simulink library "bcm"  (R2021b)
settings: Solver=VariableStepAuto  StartTime=0.0  StopTime=10.0  RelTol=1e-3
undefined symbols (not defined in the file or in its folder): ENUM_ANTITHEFT_ALARM, ENUM_ANTITHEFT_ARM, ENUM_ANTITHEFT_DISARM, ENUM_ANTITHEFT_WAIT, ENUM_GEARPOSNTOCAN_P, ENUM_PDKEYRAWLULOCK_INUNLOCK, ENUM_PDKEYRAWPS_INPS, ENUM_POWERSTA_ON, ENUM_POWERSTA_READY, ENUM_POWERSTA_STANDBY, ENUM_PWRSTASW_ON, ENUM_PWRSTASW_READY, ENUM_VEHICLETYPE_D21, ENUM_VEHICLETYPE_D31F25, ENUM_VEHICLETYPE_D31HAWD, ENUM_VEHICLETYPE_D31HRWD, ENUM_VEHICLETYPE_D31L24, FALSE, KBCM_ACCSwcPrsTmr_s, KBCM_ALMBrightnessDark_enum, KBCM_AmbBlue_enum, KBCM_AmbBreathT_ms, KBCM_AmbGreen_enum, KBCM_AmbMidPple_enum, KBCM_AmbRed_enum, KBCM_AmbTempCtrlEN_flg, KBCM_AmbTempT_s, KBCM_AmbWelModeENWait_s, KBCM_Antitheft_enum_ovrdflg, KBCM_Antitheft_enum_ovrdval, KBCM_APMDoorCtrlSta_flg_ovrdflg, KBCM_APMDoorCtrlSta_flg_ovrdval, KBCM_CmdKeepT_s, KBCM_CSWLightRstDebT_s, KBCM_CSWTurnLPRstT_s, KBCM_DelayTSW_flg, KBCM_DiagDRLOFF_flg, KBCM_DiagFLTC_mA, KBCM_DiagFMHT_s, KBCM_DiagFRTC_mA, KBCM_DiagRLTC_mA, KBCM_DiagRRTC_mA, KBCM_DrAPMRetryTimes_cnt, KBCM_DrOpenWdwOT_s, KBCM_DrOpenWdwReady_s, KBCM_ESSOffT_ms, KBCM_ESSOnT_ms, KBCM_FDCDKCReDetectT_K, KBCM_FDCDKCUSSFilterT_K, KBCM_HandleLampKeepT_s, KBCM_IVIRstHoldT_ms, KBCM_IVIRstTriggerT_ms, KBCM_ONDelayT_ms, KBCM_RAPSAbnFlashOFFT_ms, KBCM_RAPSAbnFlashONT_ms, KBCM_ReDetectT_K, KBCM_RightHandDriveEN_flg, KBCM_RLSLowSpdFilterT_s, KBCM_RmLampKeep_min, KBCM_RmLpKeyInT_s ... (+37)
libraries: simulink x447, $bdroot x11, hcu_lib x2
(part 2 of 13)

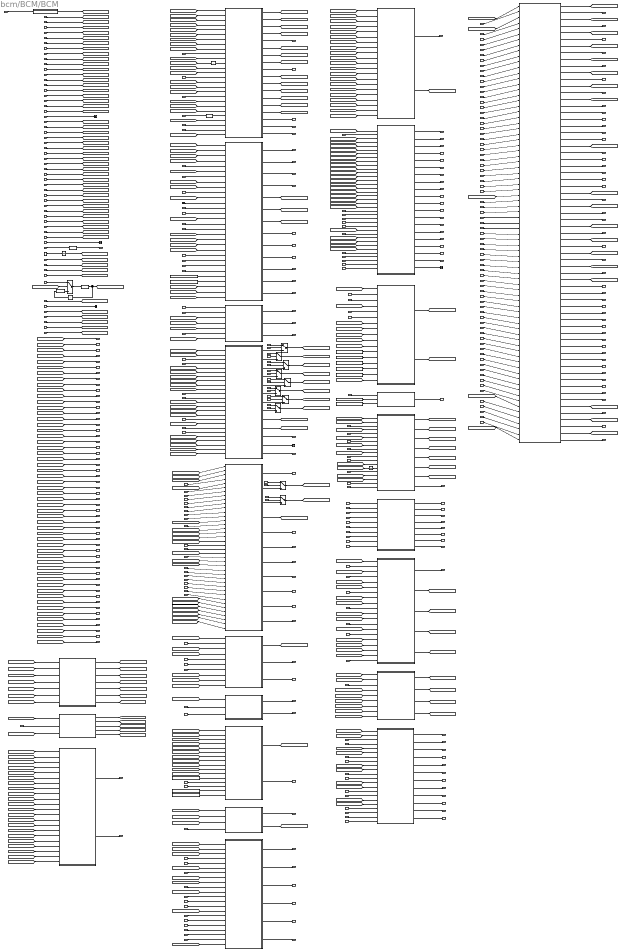
== system bcm/BCM/BCM ==
  task_time_s : Inport
  VINP_VehSpeed_kph : Inport  Port=2
  VINP_AirBagFailCmd_flg : Inport  Port=3
  VINP_ActBrkLampSta_flg : Inport  Port=4
  VINP_ESSActive_flg : Inport  Port=5
  VINP_SASAngle_Deg : Inport  Port=6
  VINP_SRRBSDWarnR_enum : Inport  Port=7
  VINP_SRRBSDWarnL_enum : Inport  Port=8
  VINP_LeftTurnReq_flg : Inport  Port=9
  VINP_RightTurnReq_flg : Inport  Port=10
  VINP_ForceLowBeam_enum : Inport  Port=11
  VINP_HazardWarningReq_flg : Inport  Port=12
  VINP_ADASACCSta_enum : Inport  Port=13
  VINP_TimeGapLevel_enum : Inport  Port=14
  VINP_SRRODASoundL_flg : Inport  Port=15
  VINP_SRRODASoundR_flg : Inport  Port=16
  VINP_SRRODAWarnL_enum : Inport  Port=17
  VINP_SRRODAWarnR_enum : Inport  Port=18
  VINP_SetUnlockSingle_flg : Inport  Port=19
  VINP_IVIStatus_flg : Inport  Port=20
  VINP_IVINightModeSta_flg : Inport  Port=21
  VINP_HeadLampSW_enum : Inport  Port=22
  VINP_RFogLampSW_flg : Inport  Port=23
  VINP_FollowMeSW_flg : Inport  Port=24
  VINP_IVIRRDefReq_flg : Inport  Port=25
  VINP_IVIWIMAINSW_flg : Inport  Port=26
  VINP_CANMsgValidIVI2_flg : Inport  Port=27
  VINP_CDLUnlockButt_flg : Inport  Port=28  OutDataTypeStr=boolean
  VINP_CDLLockButt_flg : Inport  Port=29  OutDataTypeStr=boolean
  VINP_RoomLampMode_flg : Inport  Port=30
  VINP_MFRDNBrightReq_pct : Inport  Port=31
  VINP_METERKPHCalcu_kph : Inport  Port=32
  VINP_IVIPWModeReq_enum : Inport  Port=33
  VINP_AmbLighLowBatAlertSW_flg : Inport  Port=34
  VINP_AmbLighSafetyAlertSW_flg : Inport  Port=35
  VINP_AmbLightBrightnessSet_enum : Inport  Port=36
  VINP_AmbLightDimInDarkSW_flg : Inport  Port=37
  VINP_AmbLightSW_flg : Inport  Port=38
  VINP_AmbLightWlcmLightSW_flg : Inport  Port=39
  VINP_LINKtoDRIVE_flg : Inport  Port=40
  VINP_AmbLightColorSet_enum : Inport  Port=41
  VINP_IVIPTGUSStaSW_flg : Inport  Port=42
  VINP_LDrvControlCommand_pct : Inport  Port=43
  VINP_LPasControlCommand_pct : Inport  Port=44
  VINP_LRLDControlCommand_pct : Inport  Port=45
  VINP_LRRDControlCommand_pct : Inport  Port=46
  VINP_OpenDrOpenWdoSW_flg : Inport  Port=47
  VINP_CANMsgValidIVI1_flg : Inport  Port=48
  VINP_UserSet_enum : Inport  Port=49
  VINP_TurnSwTimeSet_enum : Inport  Port=50
  VINP_IVILockSoundSWSta_flg : Inport  Port=51
  VINP_ApproachUnlockSW_flg : Inport  Port=52
  VINP_WalkawayLockSW_flg : Inport  Port=53
  VINP_IVIFrTrunkUnlockReqSta_flg : Inport  Port=54
  VINP_IVIPTGOpenHeight_enum : Inport  Port=55
  VINP_RRDefSta_flg : Inport  Port=56
  VINP_IVIStoppingUnlockSWSta_flg : Inport  Port=57
  VINP_IVIDrivingLockSWSta_flg : Inport  Port=58
  VINP_SenstivityPosition_enum : Inport  Port=59
  VINP_IVIHMICustmiKEYSta_enum : Inport  Port=60
  VINP_IVIHMICustmiFunSta_enum : Inport  Port=61
  VINP_IVIAutoWipHSpdSWCmd_flg : Inport  Port=62
  VINP_IVISWCRUndefinedSta_enum : Inport  Port=63
  VINP_HMIAutoInterLightCmd_flg : Inport  Port=64
  VINP_IVISnowModeCmd_flg : Inport  Port=65
  VINP_OFFACMode_enum : Inport  Port=66
  VINP_WlcmLightMode_enum : Inport  Port=67
  VINP_IVICarWashModeCmd_flg : Inport  Port=68
  VINP_IVIMirrorFoldedSWSta_flg : Inport  Port=69
  VINP_IVICLWinLockDrSW_flg : Inport  Port=70
  VINP_ConnDrvWdwCtrlCmd_pct : Inport  Port=71
  VINP_ConnPasWdwCtrlCmd_pct : Inport  Port=72
  VINP_ConnRLDWdwCtrlCmd_pct : Inport  Port=73
  VINP_ConnRRDWdwCtrlCmd_pct : Inport  Port=74
  VINP_HVBattSOCDis_pct : Inport  Port=75
  VINP_CSW2DimSwSta_flg : Inport  Port=76
  VINP_CSW2PassSWSta_flg : Inport  Port=77
  VINP_CSW2FWipSwSta_enum : Inport  Port=78
  VINP_CSW2FWasSwSta_enum : Inport  Port=79
  VUNP_CSW2TurnSwSta_enum : Inport  Port=80
  VINP_CSW2RWipWasSwSta_enum : Inport  Port=81
  VINP_CANMsgValidShifter2_flg : Inport  Port=82
  VINP_DrLockSta_flg : Inport  Port=83
  VINP_CSWDimSw_flg : Inport  Port=84
  VINP_CSWPassSWSta_flg : Inport  Port=85
  VINP_RLSLampSta_flg : Inport  Port=86
  VINP_CSWTurnSWSta_enum : Inport  Port=87
  VINP_RLTurnLampC_mA : Inport  Port=88
  VINP_RRTurnLampC_mA : Inport  Port=89
  VINP_FLTurnLampC_mA : Inport  Port=90
  VINP_FRTurnLampC_mA : Inport  Port=91
  VINP_MIRRORFOLDSW_flg : Inport  Port=92
  VINP_CSWFWasSWSta_enum : Inport  Port=93
  VINP_CSWFWipSWSta_enum : Inport  Port=94
  VINP_RLSRainSnrWiperCmd_enum : Inport  Port=95
  VINP_FWiperAS_flg : Inport  Port=96
  VINP_CSWRWipIntSwSta_enum : Inport  Port=97
  VINP_RWiperAS_flg : Inport  Port=98
  VINP_CSWRWasSWSta_enum : Inport  Port=99
  VINP_PTGRDILsta_enum : Inport  Port=100
  VINP_RWiperProtection_flg : Inport  Port=101
  VINP_FWiperProtection_flg : Inport  Port=102
  VINP_SWCmodeSta_flg : Inport  Port=103
  VINP_CANMsgValidDKC1_flg : Inport  Port=104
  VINP_CANMsgValidGWZoneDR1_flg : Inport  Port=105
  VINP_CANMsgValidGWZoneFR1_flg : Inport  Port=106
  VINP_PTGInnerSW2_enum : Inport  Port=107
  VINP_LDrvValWdwOpened_pct : Inport  Port=108
  VINP_LPasValWdwOpened_pct : Inport  Port=109
  VINP_LRLDValWdwOpened_pct : Inport  Port=110
  VINP_LRRDValWdwOpened_pct : Inport  Port=111
  VINP_FLHandleClose_flg : Inport  Port=112
  VINP_FRHandleClose_flg : Inport  Port=113
  VINP_RLHandleClose_flg : Inport  Port=114
  VINP_RRHandleClose_flg : Inport  Port=115
  VINP_FLTurnLPErr_flg : Inport  Port=116
  VINP_FRTurnLPErr_flg : Inport  Port=117
  VINP_RLTurnLPErr_flg : Inport  Port=118
  VINP_RRTurnLPErr_flg : Inport  Port=119
  VINP_HRLTurnLPNormalSta_flg : Inport  Port=120
  VINP_HRRTurnLPHNormalSta_flg : Inport  Port=121
  VINP_CANMsgValidZONER1_flg : Inport  Port=122
  VINP_ZRPTGRDILCmd_enum : Inport  Port=123
  VINP_BPPTGIsSetHeightSta_flg : Inport  Port=124
  VINP_PTGLeftHallPosn_cnt : Inport  Port=125
  VINP_CANMsgValidzGWLINDr1_flg : Inport  Port=126
  VINP_SWC2LRightSta_flg : Inport  Port=127
  VINP_SWC2LLeftSta_flg : Inport  Port=128
  VINP_PTGIsSetHeight_flg : Inport  Port=129
  VDKC_PDKeyAreaRAPSSta_enum : Inport  Port=130
  VINP_CANMsgValidBodyZonePS1_flg : Inport  Port=131
  VINP_LeftHallPos_cnt : Inport  Port=132
  VINP_SWC2RCustomizeSta_flg : Inport  Port=133
  VINP_BDAPMWinFOpenedSta_pct : Inport  Port=134
  VINP_BDAPMWinROpenedSta_pct : Inport  Port=135
  VINP_BPAPMWinFOpenedSta_pct : Inport  Port=136
  VINP_BPAPMWinROpenedSta_pct : Inport  Port=137
  VDKC_PDKeyAreaLockUnlock_enum : Inport  Port=138
  VDKC_PDKeyAreaPTG_enum : Inport  Port=139
  VDKC_PDKeyAreaPS_enum : Inport  Port=140
  VDKC_PCommandToBCM_enum : Inport  Port=141
  VDKC_KeyAreaSPTGSta_enum : Inport  Port=142
  VINP_PDKeyWelcome_enum : Inport  Port=143
  VINP_DKCDrvWdwCtrlCmd_pct : Inport  Port=144
  VINP_DKCPasWdwCtrlCmd_pct : Inport  Port=145
  VINP_DKCRLDWdwCtrlCmd_pct : Inport  Port=146
  VINP_DKCRRDWdwCtrlCmd_pct : Inport  Port=147
  VINP_ReDoorLock_enum : Inport  Port=148
  VINP_ReOutsideMirror_enum : Inport  Port=149
  VINP_HoodSW_flg : Inport  Port=150
  VINP_TailgateSW_flg : Inport  Port=151
  VINP_DrDoorSW_flg : Inport  Port=152
  VINP_PsDoorSW_flg : Inport  Port=153
  VINP_RLDoorSW_flg : Inport  Port=154
  VINP_RRDoorSW_flg : Inport  Port=155
  VINP_TrunkHanSW_flg : Inport  Port=156
  VINP_HazardSW_flg : Inport  Port=157
  VINP_CentralDoorLockSW_flg : Inport  Port=158
  VINP_BrakeSWGPIO_flg : Inport  Port=159
  VINP_DrSeatSta_enum : Inport  Port=160
  VPMM_PwrSta_enum : Inport  Port=161
  VTQD_ShiftGearPosn_enum : Inport  Port=162
  VTQD_CrashDetd_flg : Inport  Port=163
  VTQD_DiagHCrash_flg : Inport  Port=164
  VTQD_ReBrakeLPReq_flg : Inport  Port=165
  VINP_FDCVMCSpdCtrlModeSta_enum : Inport  Port=166
  VINP_FlashAntitheft_enum : Inport  Port=167
  VINP_FlashCountAlarm_enum : Inport  Port=168
  VINP_FlashMFSWTri_flg : Inport  Port=169
  VINP_FlashMirrorFlodPos : Inport  Port=170
  VINP_FlashFuelDoorPos : Inport  Port=171
  VINP_FlashMFRDNBrightReq_pct : Inport  Port=172
  VINP_FlashWiperFixMode_flg : Inport  Port=173
  VINP_FlashIVIPTGUSStaSW_enum : Inport  Port=174
  VINP_FlashHoodSW_flg : Inport  Port=175
  VINP_FlashTailgateSW_flg : Inport  Port=176
  VINP_FlashCTDLockSW_flg : Inport  Port=177
  VINP_FlashTailgateHDSW_flg : Inport  Port=178
  VINP_FlashAPMDoorControlSta_flg : Inport  Port=179
  VINP_FlashfUnlockSingle_flg : Inport  Port=180
  VINP_FlashAmbFunEN_enum : Inport  Port=181
  VINP_FlashAmbWelEN_enum : Inport  Port=182
  VINP_FlashAmbDimEN_enum : Inport  Port=183
  VINP_FlashAmbLinkDriSta_enum : Inport  Port=184
  VINP_FlashAmbPwrWarnEN_enum : Inport  Port=185
  VINP_FlashAmbODAEN_enum : Inport  Port=186
  VINP_FlashAmbColorSta1_enum : Inport  Port=187
  VINP_FlashAmbColorSta2_enum : Inport  Port=188
  VINP_FlashAmbColorSta3_enum : Inport  Port=189
  VINP_FlashAmbColorSta4_enum : Inport  Port=190
  VINP_FlashAmbColorSta5_enum : Inport  Port=191
  VINP_FlashAmbColorSta7_enum : Inport  Port=192
  VINP_FlashAmbBrightnessSta1_enum : Inport  Port=193
  VINP_FlashAmbBrightnessSta2_enum : Inport  Port=194
  VINP_FlashAmbBrightnessSta3_enum : Inport  Port=195
  VINP_FlashAmbBrightnessSta4_enum : Inport  Port=196
  VINP_FlashAmbBrightnessSta5_enum : Inport  Port=197
  VINP_FlashAmbBrightnessSta7_enum : Inport  Port=198
  VINP_FlashTurnSwTimeSetSta123_enum : Inport  Port=199
  VINP_FlashTurnSwTimeSetSta457_enum : Inport  Port=200
  VINP_funAuto_flg : Inport  Port=201
  VINP_DiagDRLOFF_flg : Inport  Port=202
  VINP_DiagFMHT_s : Inport  Port=203
  VINP_DiagFLTC_mA : Inport  Port=204
  VINP_DiagFRTC_mA : Inport  Port=205
  VINP_DiagRLTC_mA : Inport  Port=206
  VINP_DiagRRTC_mA : Inport  Port=207
  VINP_FlashWalkOutLkEN_enum : Inport  Port=208
  VINP_FlashWalkInUnLkEN_enum : Inport  Port=209
  VINP_FlashRmLpModeEN_enum : Inport  Port=210
  VINP_FlashLockSettingSta_enum : Inport  Port=211
  VINP_FlashFollowMeENFun_enum : Inport  Port=212
  VINP_FlashPTGUserHeight1_cnt : Inport  Port=213
  VINP_FlashPTGUserHeight2_cnt : Inport  Port=214
  VINP_FlashPTGUserHeight3_cnt : Inport  Port=215
  VINP_FlashPTGUserHeight4_cnt : Inport  Port=216
  VINP_FlashPTGUserHeight5_cnt : Inport  Port=217
  VINP_FlashPTGUserHeight7_cnt : Inport  Port=218
  VINP_FlashPTGOpenHeight12_enum : Inport  Port=219
  VINP_FlashPTGOpenHeight34_enum : Inport  Port=220
  VINP_FlashPTGOpenHeight57_enum : Inport  Port=221
  VINP_DiagWipRLSCmdCutEN_flg : Inport  Port=222
  VINP_DiagWipRLSCmdHoldEN_flg : Inport  Port=223
  VINP_DiagRLSCmdHoldTime_s : Inport  Port=224
  VINP_DiagRLSCmdCutTime_s : Inport  Port=225
  VINP_FlashACCLevelSta12_enum : Inport  Port=226
  VINP_FlashACCLevelSta34_enum : Inport  Port=227
  VINP_FlashACCLevelSta57_enum : Inport  Port=228
  VINP_FlashAutoLock_enum : Inport  Port=229
  VINP_FlashAutoUnlock_enum : Inport  Port=230
  VINP_VehicleType_enum : Inport  Port=231
  VINP_FlashHMIKey1Func_enum : Inport  Port=232
  VINP_FlashHMIKey2Func_enum : Inport  Port=233
  VINP_FlashHMIKey3Func_enum : Inport  Port=234
  VINP_FlashHMIKey4Func_enum : Inport  Port=235
  VINP_FlashHMIKey5Func_enum : Inport  Port=236
  VINP_FlashHMIKey6Func_enum : Inport  Port=237
  VINP_FlashHMIKey7Func_enum : Inport  Port=238
  VINP_FlashHMIKey8Func_enum : Inport  Port=239
  VINP_FlashAutoWipHSpdEN_flg : Inport  Port=240
  VINP_FoxPiPosLampCtrlEN_flg : Inport  Port=241
  VINP_FoxPiPosLampCtrl_flg : Inport  Port=242
  VBCM_FoxPiLBeamCtrlEN_flg : Inport  Port=243
  VBCM_FoxPiLBeamCtrl_flg : Inport  Port=244
  VBCM_FoxPiHBeamCtrlEN_flg : Inport  Port=245
  VBCM_FoxPiHBeamCtrl_flg : Inport  Port=246
  VBCM_FoxPiRDRLCtrlEN_flg : Inport  Port=247
  VBCM_FoxPiRDRLCtrl_flg : Inport  Port=248
  VBCM_FoxPiLDRLCtrlEN_flg : Inport  Port=249
  VBCM_FoxPiLDRLCtrl_flg : Inport  Port=250
  VBCM_FoxPiLTurnLPCtrlEN_flg : Inport  Port=251
  VBCM_FoxPiLTurnLPCtrl_flg : Inport  Port=252
  VBCM_FoxPiRTurnLPCtrlEN_flg : Inport  Port=253
  VBCM_FoxPiRTurnLPCtrl_flg : Inport  Port=254
  VBCM_FoxPiBkLampCtrlEN_flg : Inport  Port=255
  VBCM_FoxPiBkLampCtrl_flg : Inport  Port=256
  VBCM_FoxPiRevCtrlEN_flg : Inport  Port=257
  VBCM_FoxPiRevCtrl_flg : Inport  Port=258
  VBCM_FoxPiRrFogLpCtrlEN_flg : Inport  Port=259
  VBCM_FoxPiRrFogLpCtrl_flg : Inport  Port=260
  VINP_FoxPiAmbCtrlEN_flg : Inport  Port=261
  VINP_FoxPiAmbAreaCtrl_enum : Inport  Port=262
  VINP_FoxPiAmbColorCtrl_enum : Inport  Port=263
  VINP_FoxPiAmbBrightCtrl_enum : Inport  Port=264
  VINP_FoxPiAmbBreathCtrl_enum : Inport  Port=265
  VINP_FlashCLWinLockDrSta_enum : Inport  Port=266
  VAPM_PASDRMR_cm : Inport  Port=267
  VAPM_PASDRML_cm : Inport  Port=268
  VINP_RAPSBCMLockReqCmd_flg : Inport  Port=269
  VINP_RAPSErrWarn_enum : Inport  Port=270
  VINP_RAPSBCMLamp_enum : Inport  Port=271
  VINP_APSStaSystem_enum : Inport  Port=272
  VTPM_TPMSTLCmd_flg : Inport  Port=273
  VTHC_Z1UP_flg : Inport  Port=274
  VTHC_Z2UP_flg : Inport  Port=275
  VTHC_Z1DN_flg : Inport  Port=276
  VTHC_Z2DN_flg : Inport  Port=277
  VDDM_HVRlyOpCFS_flg : Inport  Port=278
  VDDM_MCUActCFS_flg : Inport  Port=279
  APM_Door : Subsystem
  Amb : Subsystem
  AntiTheft : Subsystem
  BCM_WAKE_MODULE : Subsystem
  BCM_Window_Control : Subsystem
  CSW : Subsystem
  CenterDoorLock : Subsystem
  Constant10 : Constant  Value=KBCM_DelayTSW_flg
  Constant11 : Constant  Value=KBCM_ReDetectT_K
  Constant12 : Constant  Value=KBCM_SPTGDetectT_sec
  Constant13 : Constant  Value=KBCM_SPTGLeave_flg
  Constant14 : Constant  Value=KBCM_RmLampKeep_min
  Constant15 : Constant  Value=KBCM_SPTGWaitDKC_sec
  Constant17 : Constant
  Constant18 : Constant  Value=KBCM_RmLpKeyInT_s
  Constant19 : Constant  Value=KBCM_RmLpKeyMissT_s
  Constant6 : Constant  Value=KBCM_CmdKeepT_s  OutDataTypeStr=single
  Constant7 : Constant  Value=KBCM_HandleLampKeepT_s  OutDataTypeStr=single
  Constant8 : Constant  Value=KBCM_IVIRstHoldT_ms
  Constant9 : Constant  Value=KBCM_IVIRstTriggerT_ms
  DID Judgement : Subsystem
  Data Type Conversion : DataTypeConversion  OutDataTypeStr=uint8
  Data Type Conversion1 : DataTypeConversion  OutDataTypeStr=boolean
  Data Type Conversion2 : DataTypeConversion  OutDataTypeStr=boolean
  Detect Increase : simulink/Logic and Bit Operations/Detect Increase  vinit=0.0  OutDataTypeStr=boolean
  Dimmer : Subsystem
  ExteriorLight : Subsystem
  FlasherSignal : Subsystem
  FoxtronPiOutput : Subsystem
  Ground : Ground
  HMI_Custom_Button : Subsystem
  IVI Reset : Subsystem
  PTG : Subsystem
  Personal_Setting : Subsystem
  PowerMirror : Subsystem
  RearDefogger : Subsystem
  RoomLamp : Subsystem
  Switch{,1..10} (11 alike) : Switch  Criteria=u2 > Threshold
  Tailgate : Subsystem
  Terminator{,1..2,7..8} (5 alike) : Terminator
  Unit Delay{,1..3} (4 alike) : UnitDelay  SampleTime=-1  HasFrameUpgradeWarning=on
  Vehicle Type Diff Fun : Subsystem
  Verify : Subsystem
  WasherWiper : Subsystem
  Window_Control_Sig_Combine : Subsystem
  VBCM_AntitheftSta_enum : Outport
  VBCM_TailgateRemote_enum : Outport  Port=2
  VBCM_HornCtrl_flg : Outport  Port=3
  VBCM_AllDoorSW_flg : Outport  Port=4
  VBCM_BCMDoorLockSta_flg : Outport  Port=5
  VBCM_AntitheftSeatFlod_flg : Outport  Port=6
  VBCM_HoodSW_flg : Outport  Port=7
  VBCM_TailgateSW_flg : Outport  Port=8
  VBCM_DrDoorSW_flg : Outport  Port=9
  VBCM_PsDoorSW_flg : Outport  Port=10
  VBCM_RLDoorSW_flg : Outport  Port=11
  VBCM_RRDoorSW_flg : Outport  Port=12
  VBCM_LockSetting_flg : Outport  Port=13
  VBCM_FrChargingDoorCtrl_enum : Outport  Port=14
  VBCM_RrChargingDoorCtrl_enum : Outport  Port=15
  VBCM_CrashSDetd_flg : Outport  Port=16
  VBCM_CTDCtrl_enum : Outport  Port=17
  VBCM_DoorLockIND_flg : Outport  Port=18
  VBCM_CTDLockSW_flg : Outport  Port=19
  VBCM_Dimmer_pct : Outport  Port=20
  VBCM_DimmerEN_flg : Outport  Port=21
  VBCM_PosLamp_flg : Outport  Port=22
  VBCM_LBeam_flg : Outport  Port=23
  VBCM_HBeam_flg : Outport  Port=24
  VBCM_RrFogLamp_flg : Outport  Port=25
  VBCM_BrakeLamp_flg : Outport  Port=26
  VBCM_ReverseLamp_flg : Outport  Port=27
  VBCM_LDRL_flg : Outport  Port=28
  VBCM_RDRL_flg : Outport  Port=29
  VBCM_LBSD_flg : Outport  Port=30
  VBCM_RBSD_flg : Outport  Port=31
  VBCM_HazardSW_flg : Outport  Port=32
  VBCM_LTurnLP_flg : Outport  Port=33
  VBCM_RTurnLP_flg : Outport  Port=34
  VBCM_BCMBuzzerReq_flg : Outport  Port=35
  VBCM_MirrorCtrl_enum : Outport  Port=36
  VBCM_MirrorDefog_flg : Outport  Port=37
  VBCM_RrDefog_flg : Outport  Port=38
  VBCM_RoomLampH_flg : Outport  Port=39
  VBCM_RoomLampL_flg : Outport  Port=40
  VBCM_TrunkRel_flg : Outport  Port=41
  VBCM_TailgateHDSW_flg : Outport  Port=42
  VBCM_FWiperL_flg : Outport  Port=43
  VBCM_FWiperH_flg : Outport  Port=44
  VBCM_RWiper_flg : Outport  Port=45
  VBCM_WasherCtrl_enum : Outport  Port=46
  VBCM_WiperFixMode_flg : Outport  Port=47
  VBCM_SleepReq_flg : Outport  Port=48
  VBCM_AmbLightBreath1_enum : Outport  Port=49
  VBCM_AmbLightBreath2_enum : Outport  Port=50
  VBCM_AmbLightBreath3_enum : Outport  Port=51
  VBCM_AmbLightBreath4_enum : Outport  Port=52
  VBCM_AmbLightBreath5_enum : Outport  Port=53
  VBCM_AmbLightBreath6_enum : Outport  Port=54
  VBCM_AmbLightBrightness1_enum : Outport  Port=55
  VBCM_AmbLightBrightness2_enum : Outport  Port=56
  VBCM_AmbLightBrightness3_enum : Outport  Port=57
  VBCM_AmbLightBrightness4_enum : Outport  Port=58
  VBCM_AmbLightBrightness5_enum : Outport  Port=59
  VBCM_AmbLightBrightness6_enum : Outport  Port=60
  VBCM_AmbLightColor1_enum : Outport  Port=61
  VBCM_AmbLightColor2_enum : Outport  Port=62
  VBCM_AmbLightColor3_enum : Outport  Port=63
  VBCM_AmbLightColor4_enum : Outport  Port=64
  VBCM_AmbLightColor5_enum : Outport  Port=65
  VBCM_AmbLightColor6_enum : Outport  Port=66
  VBCM_LampPwr_flg : Outport  Port=67
  VBCM_SPTGDet_flg : Outport  Port=68
  VBCM_APSOpenPTG_flg : Outport  Port=69
  VBCM_FollowMe_flg : Outport  Port=70
  VBCM_IVIRST_flg : Outport  Port=71
  VBCM_CountAlarm_enum : Outport  Port=72
  VBCM_MFSWTri_flg : Outport  Port=73
  VBCM_MirrorFlodPos_flg : Outport  Port=74
  VBCM_FuelDoorPos_flg : Outport  Port=75
  VBCM_MFRDNBrightReq_pct : Outport  Port=76
  VBCM_PTGInnerSW2_enum : Outport  Port=77
  VBCM_DiagHCrash_flg : Outport  Port=78
  VBCM_DiagFLTS_flg : Outport  Port=79
  VBCM_DiagFRTS_flg : Outport  Port=80
  VBCM_DiagRLTS_flg : Outport  Port=81
  VBCM_DiagRRTS_flg : Outport  Port=82
  VBCM_DrvWdwCtrlCmd_pct : Outport  Port=83
  VBCM_PasWdwCtrlCmd_pct : Outport  Port=84
  VBCM_DrRWdwCtrlCmd_pct : Outport  Port=85
  VBCM_PsRWdwCtrlCmd_pct : Outport  Port=86
  VBCM_APMDoorControlSta_flg : Outport  Port=87
  VBCM_AmbFunEN_flg : Outport  Port=88
  VBCM_AmbWelEN_flg : Outport  Port=89
  VBCM_AmbDimEN_flg : Outport  Port=90
  VBCM_AmbLinkDriSta_flg : Outport  Port=91
  VBCM_AmbPwrWarnEN_flg : Outport  Port=92
  VBCM_AmbODAEN_flg : Outport  Port=93
  VBCM_AmbColorSta_enum : Outport  Port=94
  VBCM_AmbBrightSta_enum : Outport  Port=95
  VBCM_LockAlarm_enum : Outport  Port=96
  VBCM_ATCtrl_enum : Outport  Port=97
  VBCM_fUnlockSingle_flg : Outport  Port=98
  VBCM_UserNow_enum : Outport  Port=99
  VBCM_AmbFunENFlash_enum : Outport  Port=100
  VBCM_AmbWelENFlash_enum : Outport  Port=101
  VBCM_AmbDimENFlash_enum : Outport  Port=102
  VBCM_AmbLinkDriStaFlash_enum : Outport  Port=103
  VBCM_AmbPwrWarnENFlash_enum : Outport  Port=104
  VBCM_AmbODAENFlash_enum : Outport  Port=105
  VBCM_AmbColorSta1_enum : Outport  Port=106
  VBCM_AmbColorSta2_enum : Outport  Port=107
  VBCM_AmbColorSta3_enum : Outport  Port=108
  VBCM_AmbColorSta4_enum : Outport  Port=109
  VBCM_AmbColorSta5_enum : Outport  Port=110
  VBCM_AmbColorSta7_enum : Outport  Port=111
  VBCM_AmbBrightnessSta1_enum : Outport  Port=112
  VBCM_AmbBrightnessSta2_enum : Outport  Port=113
  VBCM_AmbBrightnessSta3_enum : Outport  Port=114
  VBCM_AmbBrightnessSta4_enum : Outport  Port=115
  VBCM_AmbBrightnessSta5_enum : Outport  Port=116
  VBCM_AmbBrightnessSta7_enum : Outport  Port=117
  VBCM_HazardIND_flg : Outport  Port=118
  VBCM_DimSwSta_flg : Outport  Port=119
  VBCM_PassSWSta_flg : Outport  Port=120
  VBCM_FWipSwSta_enum : Outport  Port=121
  VBCM_FWasSwSta_enum : Outport  Port=122
  VBCM_TurnSwSta_enum : Outport  Port=123
  VBCM_TurnSwTSetSta_enum : Outport  Port=124
  VBCM_SPTGENFun_flg : Outport  Port=125
  VBCM_SPTGENFunMem_enum : Outport  Port=126
  VBCM_OutMode_enum : Outport  Port=127
  VBCM_TurnSwTimeSetSta123_enum : Outport  Port=128
  VBCM_TurnSwTimeSetSta457_enum : Outport  Port=129
  VBCM_FDLHandleLampCmd_flg : Outport  Port=130
  VBCM_FDRHandleLampCmd_flg : Outport  Port=131
  VBCM_FDHandleCmd_enum : Outport  Port=132
  VBCM_HBeamADB_flg : Outport  Port=133
  VBCM_WalkInUnLkENMem_enum : Outport  Port=134
  VBCM_WalkOutLkENMem_enum : Outport  Port=135
  VBCM_RmLpModeENMem_enum : Outport  Port=136
  VBCM_LockSettingStaMem_enum : Outport  Port=137
  VBCM_FollowMeENMem_enum : Outport  Port=138
  VBCM_WalkInUnLkEnFunSta_flg : Outport  Port=139
  VBCM_WalkOutLkEnFunSta_flg : Outport  Port=140
  VBCM_RmLpModeENFunSta_flg : Outport  Port=141
  VBCM_FollowMeENFunSta_flg : Outport  Port=142
  VBCM_HoodRelCmd_flg : Outport  Port=143
  VBCM_WelcomeLight_enum : Outport  Port=144
  VBCM_PTGOpenHeightSta_enum : Outport  Port=145
  VBCM_UserHeightSet_cnt : Outport  Port=146
  VBCM_PTGUserHeight1_cnt : Outport  Port=147
  VBCM_PTGUserHeight2_cnt : Outport  Port=148
  VBCM_PTGUserHeight3_cnt : Outport  Port=149
  VBCM_PTGUserHeight4_cnt : Outport  Port=150
  VBCM_PTGUserHeight5_cnt : Outport  Port=151
  VBCM_PTGUserHeight7_cnt : Outport  Port=152
  VBCM_PTGOpenHeight12_enum : Outport  Port=153
  VBCM_PTGOpenHeight34_enum : Outport  Port=154
  VBCM_PTGOpenHeight57_enum : Outport  Port=155
  VBCM_SenstivityPosnCmd_enum : Outport  Port=156
  VBCM_TimeGapLevelSta_enum : Outport  Port=157
  VBCM_ACCLevelMem12_enum : Outport  Port=158
  VBCM_ACCLevelMem34_enum : Outport  Port=159
  VBCM_ACCLevelMem57_enum : Outport  Port=160
  VBCM_LRightStaCmd_flg : Outport  Port=161
  VBCM_LLeftStaCmd_flg : Outport  Port=162
  VBCM_AutoLockSta_flg : Outport  Port=163
  VBCM_AutoLockMem_enum : Outport  Port=164
  VBCM_AutoUnlockSta_flg : Outport  Port=165
  VBCM_AutoUnlockMem_enum : Outport  Port=166
  VBCM_HMIKey1FuncSta_enum : Outport  Port=167
  VBCM_HMIKey2FuncSta_enum : Outport  Port=168
  VBCM_HMIKey3FuncSta_enum : Outport  Port=169
  VBCM_HMIKey4FuncSta_enum : Outport  Port=170
  VBCM_HMIKey5FuncSta_enum : Outport  Port=171
  VBCM_HMIKey6FuncSta_enum : Outport  Port=172
  VBCM_HMIKey7FuncSta_enum : Outport  Port=173
  VBCM_HMIKey8FuncSta_enum : Outport  Port=174
  VBCM_AutoWipHSpdENSta_flg : Outport  Port=175
  VBCM_DrvWdwReqAP_enum : Outport  Port=176
  VBCM_PasWdwReqAP_enum : Outport  Port=177
  VBCM_DrRWdwReqAP_enum : Outport  Port=178
  VBCM_PsRWdwReqAP_enum : Outport  Port=179
  VBCM_CLWinLockDrSta_flg : Outport  Port=180
  VBCM_CLWinLockDrStaMem_enum : Outport  Port=181
  VBCM_WinLFOpenedSta_pct : Outport  Port=182
  VBCM_WinRFOpenedSta_pct : Outport  Port=183
  VBCM_WinLROpenedSta_pct : Outport  Port=184
  VBCM_WinRROpenedSta_pct : Outport  Port=185
  VBCM_FoxPiSwitchSta_enum : Outport  Port=186
  VBCM_FoxPiLampSta_enum : Outport  Port=187
  wires:
  VPMM_PwrSta_enum/1 -> [VPMM_PwrSta_enum]
  VINP_TailgateSW_flg/1 -> [VINP_TailgateSW_flg]
  VINP_ReDoorLock_enum/1 -> AntiTheft/10(VINP_ReDoorLock_enum)
  VINP_VehSpeed_kph/1 -> [VINP_VehSpeed_kph]
  AntiTheft/4(VBCM_AntitheftSta_enum) -> [VBCM_AntitheftSta_enum]
  AntiTheft/5(VBCM_TailgateRemote_enum) -> VBCM_TailgateRemote_enum/1
  AntiTheft/6(VBCM_HornCtrl_flg) -> [VBCM_HornCtrl_flg]
  AntiTheft/7(VBCM_AllDoorSW_flg) -> [VBCM_AllDoorSW_flg]
  AntiTheft/9(VBCM_AntitehftSeatFlod_flg) -> VBCM_AntitheftSeatFlod_flg/1
  AntiTheft/8(VBCM_BCMDoorLockSta_flg) -> [VBCM_BCMDoorLockSta_flg]
  AntiTheft/1(VBCM_ATCtrl_enum) -> [VBCM_ATCtrl_enum]
  AntiTheft/2(VBCM_ATActCtrl_enum) -> [VBCM_ATActCtrl_enum]
  AntiTheft/3(VBCM_ATAlarm_flg) -> [VBCM_ATAlarm_flg]
  [VBCM_AllDoorSW_flg] -> CenterDoorLock/4(VBCM_AllDoorSW_flg)
  [VBCM_AntitheftSta_enum] -> CenterDoorLock/3(VBCM_AntitheftSta_enum)
  [VPMM_PwrSta_enum] -> CenterDoorLock/6(VPMM_PwrSta_enum)
  CenterDoorLock/6(VBCM_fVIGHandle_flg) -> [VBCM_fVIGHandle_flg]
  VTQD_DiagHCrash_flg/1 -> CenterDoorLock/5(VTQD_DiagHCrash_flg)
  VINP_CentralDoorLockSW_flg/1 -> CenterDoorLock/7(VINP_CentralDoorLockSW_flg)
  [VBCM_BCMDoorLockSta_flg] -> CenterDoorLock/8(VBCM_BCMDoorLockSta_flg)
  [VBCM_ATActCtrl_enum] -> CenterDoorLock/9(VBCM_ATActCtrl_enum)
  [VINP_VehSpeed_kph] -> CenterDoorLock/11(VINP_VehSpeed_kph)
  VINP_AirBagFailCmd_flg/1 -> CenterDoorLock/10(VINP_AirBagFailCmd_flg)
  CenterDoorLock/1(VBCM_FrChargingDoorCtrl_enum) -> VBCM_FrChargingDoorCtrl_enum/1
  CenterDoorLock/2(VBCM_RrChargingDoorCtrl_enum) -> VBCM_RrChargingDoorCtrl_enum/1
  CenterDoorLock/3(VBCM_CrashDetd_flg) -> VBCM_CrashSDetd_flg/1
  CenterDoorLock/4(VBCM_CTDCtrl_enum) -> VBCM_CTDCtrl_enum/1
  CenterDoorLock/5(DoorLockIND) -> [VBCM_DoorLockIND_flg]
  VINP_MFRDNBrightReq_pct/1 -> Dimmer/1(VINP_MFRDNBrightReq_pct)
  VINP_IVIStatus_flg/1 -> Dimmer/2(VINP_IVIStatus_flg)
  Dimmer/1(VBCM_Dimmer_pct) -> VBCM_Dimmer_pct/1
  Dimmer/2(VBCM_DimmerEN_flg) -> VBCM_DimmerEN_flg/1
  [VBCM_PosLamp_flg] -> Dimmer/4(VBCM_PosLamp_flag)
  [VPMM_PwrSta_enum] -> PowerMirror/1(VPMM_PwrSta_enum)
  VINP_MIRRORFOLDSW_flg/1 -> PowerMirror/2(VINP_MIRRORFOLDSW_flg)
  [VINP_VehSpeed_kph] -> PowerMirror/3(VINP_VehSpeed_kph)
  [VBCM_ATActCtrl_enum] -> PowerMirror/4(VBCM_ATActCtrl_enum)
  PowerMirror/1(VBCM_MirrorCtrl_enum) -> [VBCM_MirrorCtrl_enum]
  [VPMM_PwrSta_enum] -> RearDefogger/1(VPMM_PwrSta_enum)
  VINP_RRDefSta_flg/1 -> RearDefogger/2(VINP_RRDefSta_flg)
  VINP_IVIRRDefReq_flg/1 -> RearDefogger/3(VINP_IVIRRDefReq_flg)
  RearDefogger/1(VBCM_MirrorDefog_flg) -> VBCM_MirrorDefog_flg/1
  RearDefogger/2(VBCM_RrDefog_flg) -> VBCM_RrDefog_flg/1
  [VPMM_PwrSta_enum] -> RoomLamp/2(VPMM_PwrSta_enum)
  [VBCM_BCMDoorLockSta_flg] -> RoomLamp/3(VBCM_BCMDoorLockSta_flg)
  [VBCM_AllDoorSW_flg] -> RoomLamp/4(VBCM_AllDoorSW_flg)
  [VBCM_AntitheftSta_enum] -> RoomLamp/5(VBCM_AntitheftSta_enum)
  [VPMM_PwrSta_enum] -> Tailgate/1(VPMM_PwrSta_enum)
  [VINP_VehSpeed_kph] -> Tailgate/2(VINP_VehSpeed_kph)
  [VBCM_BCMDoorLockSta_flg] -> Tailgate/3(VBCM_BCMDoorLockSta_flg)
  VINP_TrunkHanSW_flg/1 -> Tailgate/4(VINP_TrunkHandleSwSG08_flg)
  Tailgate/1(VBCM_TrunkRel_flg) -> VBCM_TrunkRel_flg/1
  Unit Delay/1 -> AntiTheft/12(VBCM_fVIGHandle_flg)
  [VBCM_fVIGHandle_flg] -> Unit Delay/1
  VINP_CDLUnlockButt_flg/1 -> CenterDoorLock/13(VINP_CDLUnlockButt_flg)
  VINP_CDLLockButt_flg/1 -> CenterDoorLock/14(VINP_CDLLockButt_flg)
  AntiTheft/10(VBCM_HoodSW_flg) -> [VBCM_HoodSW_flg]
  AntiTheft/11(VBCM_TailgateSW_flg) -> [VBCM_TailgateSW_flg]
  CenterDoorLock/7(VBCM_CTDLockSW_flg) -> [VBCM_CTDLockSW_flg]
  Tailgate/2(VBCM_TailgateHDSW_flg) -> [VBCM_TailgateHDSW_flg]
  VINP_CANMsgValidIVI2_flg/1 -> [VINP_CANMsgValidIVI2_flg]
  [VINP_TailgateSW_flg] -> RoomLamp/11(VINP_TailgateSW_flg)
  CenterDoorLock/9(VBCM_DiagHCrash_flg) -> VBCM_DiagHCrash_flg/1
  [VBCM_ATCtrl_enum] -> FlasherSignal/1(VBCM_ATCtrl_enum)
  [VBCM_ATAlarm_flg] -> FlasherSignal/2(VBCM_ATAlarm_flg)
  [VPMM_PwrSta_enum] -> FlasherSignal/3(VPMM_PwrSta_enum)
  VINP_HazardSW_flg/1 -> FlasherSignal/4(VINP_HazardSW_flg)
  VINP_RLTurnLampC_mA/1 -> FlasherSignal/6(VINP_RLTurnLampC_mA)
  VINP_RRTurnLampC_mA/1 -> FlasherSignal/7(VINP_RRTurnLampC_mA)
  VINP_FLTurnLampC_mA/1 -> FlasherSignal/8(VINP_FLTurnLampC_mA)
  VINP_FRTurnLampC_mA/1 -> FlasherSignal/9(VINP_FRTurnLampC_mA)
  VINP_PTGRDILsta_enum/1 -> FlasherSignal/10(VINP_PTGRDILsta_enum)
  VINP_ESSActive_flg/1 -> FlasherSignal/11(VINP_ESSActive_flg)
  VINP_LeftTurnReq_flg/1 -> FlasherSignal/12(VINP_LeftTurnReq_flg)
  VINP_RightTurnReq_flg/1 -> FlasherSignal/13(VINP_RightTurnReq_flg)
  VINP_HazardWarningReq_flg/1 -> FlasherSignal/15(HazardWarningReq)
  FlasherSignal/1(VBCM_HazardSW_flg) -> VBCM_HazardSW_flg/1
  task_time_s/1 -> [task_time_s]
  [VBCM_HoodSW_flg] -> BCM_WAKE_MODULE/1(VBCM_HoodSW_flg)
  [VBCM_TailgateSW_flg] -> BCM_WAKE_MODULE/2(VBCM_TailgateSW_flg)
  [VBCM_CTDLockSW_flg] -> BCM_WAKE_MODULE/3(VBCM_CTDLockSW_flg)
  [VBCM_TailgateHDSW_flg] -> BCM_WAKE_MODULE/4(VBCM_TailgateHDSW_flg)
  [VBCM_AntitheftSta_enum] -> BCM_WAKE_MODULE/5(VBCM_AntitheftSta_enum)
  [VBCM_AllDoorSW_flg] -> BCM_WAKE_MODULE/6(VBCM_AllDoorSW_flg)
  [VBCM_HornCtrl_flg] -> BCM_WAKE_MODULE/7(VBCM_HornCtrl_flg)
  [VBCM_DoorLockIND_flg] -> BCM_WAKE_MODULE/8(VBCM_DoorLockIND_flg)
  [VINP_BrakeSWGPIO_flg] -> BCM_WAKE_MODULE/9(VINP_BrakeSWGPIO_flg)
  [VBCM_PosLamp_flg] -> BCM_WAKE_MODULE/10(VBCM_PosLamp_flg)
  [VBCM_LBSD_flg] -> BCM_WAKE_MODULE/11(VBCM_LBSD_flg)
  [VBCM_RBSD_flg] -> BCM_WAKE_MODULE/12(VBCM_RBSD_flg)
  [VBCM_RTurnLP_flg] -> BCM_WAKE_MODULE/14(VBCM_RTurnLP_flg)
  [VBCM_LTurnLP_flg] -> BCM_WAKE_MODULE/13(VBCM_LTurnLP_flg)
  [VBCM_MirrorCtrl_enum] -> BCM_WAKE_MODULE/15(VBCM_MirrorCtrl_enum)
  [VBCM_RoomLampH_flg] -> BCM_WAKE_MODULE/16(VBCM_RoomLampH_flg)
  [task_time_s] -> BCM_WAKE_MODULE/17(task_time_s)
  BCM_WAKE_MODULE/1(VBCM_SleepReq_flg) -> VBCM_SleepReq_flg/1
  [VPMM_PwrSta_enum] -> ExteriorLight/2(VPMM_PwrSta_enum)
  VINP_ForceLowBeam_enum/1 -> ExteriorLight/17(VINP_ForceLowBeam_enum)
  VTQD_ReBrakeLPReq_flg/1 -> ExteriorLight/19(VTQD_ReBrakeLPReq_flg)
  VINP_METERKPHCalcu_kph/1 -> ExteriorLight/20(VINP_METERKPHCalcu_kph)
  VINP_SRRBSDWarnR_enum/1 -> [VINP_SRRBSDWarnR_enum]
  VINP_SRRODASoundL_flg/1 -> [VINP_SRRODASoundL_flg]
  VINP_SRRODASoundR_flg/1 -> [VINP_SRRODASoundR_flg]
  VINP_ActBrkLampSta_flg/1 -> ExteriorLight/12(VINP_ActBrkLampSta_flg)
  VINP_RLSLampSta_flg/1 -> ExteriorLight/11(VINP_RLSLampSta_flg)
  VINP_RFogLampSW_flg/1 -> ExteriorLight/4(VINP_RFogLampSW_flg)
  VINP_HeadLampSW_enum/1 -> ExteriorLight/3(VINP_HeadLampSW_enum)
  [VINP_CANMsgValidIVI2_flg] -> ExteriorLight/18(VINP_CANMsgValidIVI2_flg)
  [VBCM_ATCtrl_enum] -> ExteriorLight/10(VBCM_ATCtrl_enum)
  [VBCM_OutMode_enum] -> ExteriorLight/9(VBCM_OutMode_enum)
  VINP_BrakeSWGPIO_flg/1 -> [VINP_BrakeSWGPIO_flg]
  [VINP_BrakeSWGPIO_flg] -> ExteriorLight/5(VINP_BrakeSWGPIO_flg)
  ExteriorLight/10(VBCM_RBSD_flg) -> [VBCM_RBSD_flg]
  ExteriorLight/9(VBCM_LBSD_flg) -> [VBCM_LBSD_flg]
  [VINP_TailgateSW_flg] -> AntiTheft/4(VINP_TailgateSW_flg)
  [VINP_DrDoorSW_flg] -> AntiTheft/5(VINP_DrDoorSW_flg)
  [VINP_VehSpeed_kph] -> AntiTheft/11(VINP_VehSpeed_kph)
  VINP_DrDoorSW_flg/1 -> [VINP_DrDoorSW_flg]
  [VPMM_PwrSta_enum] -> AntiTheft/2(VPMM_PwrSta_enum)
  VINP_IVINightModeSta_flg/1 -> [VINP_IVINightModeSta_flg]
  [VINP_IVINightModeSta_flg] -> Dimmer/3(VINP_IVINightModeSta_flg)
  [VBCM_AntitheftSta_enum] -> VBCM_AntitheftSta_enum/1
  [VINP_CANMsgValidIVI2_flg] -> Dimmer/5(VINP_CANMsgValidIVI2_flg)
  VINP_ReOutsideMirror_enum/1 -> PowerMirror/5(VINP_ReOutsideMirror_enum)
  BCM_WAKE_MODULE/2(VBCM_WakeUp_flg) -> [VBCM_WakeUp_flg]
  VINP_FlashAntitheft_enum/1 -> Verify/1(VINP_FlashAntitheft_enum)
  Verify/1(VBCM_FlashAntitheft_enum) -> [VBCM_FlashAntitheft_enum]  "VBCM_FlashAntitheft_enum"
  [VPMM_PwrSta_enum] -> WasherWiper/9(VPMM_PwrSta_enum)
  [VINP_CANMsgValidIVI2_flg] -> WasherWiper/11(VINP_CANMsgValidIVI2_flg)
  VINP_FWiperProtection_flg/1 -> WasherWiper/13(VINP_FWiperProtection_flg)
  VINP_RLSRainSnrWiperCmd_enum/1 -> WasherWiper/4(VINP_RLSRainSnrWiperCmd_enum)
  VINP_FWiperAS_flg/1 -> WasherWiper/5(VINP_FWiperAS_flg)
  VINP_RWiperAS_flg/1 -> WasherWiper/7(VINP_RWiperAS_flg)
  VINP_IVIWIMAINSW_flg/1 -> WasherWiper/10(VINP_IVIWIMAINSW_flg)
  VINP_RWiperProtection_flg/1 -> WasherWiper/12(VINP_RWiperProtection_flg)
  WasherWiper/1(VBCM_FrWiperL_flg) -> VBCM_FWiperL_flg/1
  WasherWiper/2(VBCM_FrWiperH_flg) -> VBCM_FWiperH_flg/1
  WasherWiper/3(VBCM_RrWiper_flg) -> VBCM_RWiper_flg/1
  WasherWiper/4(VBCM_WasherCtrl_enum) -> VBCM_WasherCtrl_enum/1
  WasherWiper/5(VBCM_WiperFixMode_flg) -> VBCM_WiperFixMode_flg/1
  [VBCM_APSOpenPTG_flg] -> AntiTheft/14(VINP_APSOpenPTG_flg)
  [VBCM_SPTGDet_flg] -> FlasherSignal/14(VINP_SPTGDet_flg)
  VTQD_ShiftGearPosn_enum/1 -> [VTQD_ShiftGearPosn_enum]
  [VTQD_ShiftGearPosn_enum] -> ExteriorLight/8(VTQD_ShiftGearPosn_enum)
  VDKC_PCommandToBCM_enum/1 -> [VDKC_PCommandToBCM_enum]
  [VDKC_PCommandToBCM_enum] -> AntiTheft/1(VINP_PCommandToBCM_enum)
  Constant8/1 -> IVI Reset/2(KBCM_IVIRstHoldT_ms)
  Constant9/1 -> IVI Reset/3(KBCM_IVIRstTriggerT_ms)
  VINP_SWCmodeSta_flg/1 -> IVI Reset/1(VINP_SWCmodeSta_flg)
  IVI Reset/1(VBCM_IVIRST_flg) -> VBCM_IVIRST_flg/1
  ExteriorLight/11(VBCM_FollowMe_flg) -> VBCM_FollowMe_flg/1
  VDDM_MCUActCFS_flg/1 -> FlasherSignal/21(VDDM_MCUActCFS_flg)
  VDDM_HVRlyOpCFS_flg/1 -> FlasherSignal/20(VDDM_HVRlyOpCFS_flg)
  Constant14/1 -> RoomLamp/12(KBCM_RmLampKeep_min)
  VINP_FlashMFSWTri_flg/1 -> PowerMirror/6(EEP_MFSWTri_flg)
  VINP_FlashMirrorFlodPos/1 -> PowerMirror/7(EEP_MirrorFlodPos)
  PowerMirror/2(MFSWTri) -> VBCM_MFSWTri_flg/1
  PowerMirror/3(MirrorFlodPos) -> VBCM_MirrorFlodPos_flg/1
  VINP_FlashFuelDoorPos/1 -> CenterDoorLock/16(EEP_FuelDoorPos)
  CenterDoorLock/8(VBCM_FuelDoorPos_flg) -> VBCM_FuelDoorPos_flg/1
  VINP_FlashCountAlarm_enum/1 -> AntiTheft/15(VINP_FlashCountAlarm_enum)
  AntiTheft/16(VBCM_CountAlarm_enum) -> VBCM_CountAlarm_enum/1
  VINP_FlashMFRDNBrightReq_pct/1 -> Dimmer/6(EEP_MFRDNBrightReq)
  VINP_FlashWiperFixMode_flg/1 -> WasherWiper/14(VINP_FlashWiperFixMode)
  Dimmer/3(VBCM_MFRDNBrightReq_pct) -> VBCM_MFRDNBrightReq_pct/1
  Constant17/1 -> Unit Delay1/1
  [BCMInitial] -> WasherWiper/15(BCMInitial)
  [BCMInitial] -> Dimmer/7(BCMInitial)
  Data Type Conversion/1 -> VBCM_PTGInnerSW2_enum/1  "VBCM_PTGInnerSW2_enum"
  VINP_PTGInnerSW2_enum/1 -> Data Type Conversion/1
  VINP_FlashHoodSW_flg/1 -> [VINP_FlashHoodSW_flg]
  VINP_FlashTailgateSW_flg/1 -> [VINP_FlashTailgateSW_flg]
  VINP_FlashCTDLockSW_flg/1 -> [VINP_FlashCTDLockSW_flg]
  VINP_FlashTailgateHDSW_flg/1 -> [VINP_FlashTailgateHDSW_flg]
  [VINP_FlashHoodSW_flg] -> BCM_WAKE_MODULE/18(VINP_FlashHoodSW_flg)
  [VINP_FlashTailgateSW_flg] -> BCM_WAKE_MODULE/19(VINP_FlashTailgateSW_flg)
  [VINP_FlashCTDLockSW_flg] -> BCM_WAKE_MODULE/20(VINP_FlashCTDLockSW_flg)
  [VINP_FlashTailgateHDSW_flg] -> BCM_WAKE_MODULE/21(VINP_FlashTailgateHDSW_flg)
  APM_Door/1(VBCM_APMDoorControlSta_flg) -> VBCM_APMDoorControlSta_flg/1
  VINP_PsDoorSW_flg/1 -> [VINP_PsDoorSW_flg]
  VINP_RLDoorSW_flg/1 -> [VINP_RLDoorSW_flg]
  VINP_RRDoorSW_flg/1 -> [VINP_RRDoorSW_flg]
  [VINP_PsDoorSW_flg] -> AntiTheft/6(VINP_PsDoorSW_flg)
  [VINP_RLDoorSW_flg] -> AntiTheft/7(VINP_RLDoorSW_flg)
  [VINP_RRDoorSW_flg] -> AntiTheft/8(VINP_RRDoorSW_flg)
  VINP_CANMsgValidGWZoneDR1_flg/1 -> [VINP_CANMsgValidGWZoneDR1_flg]
  VINP_CANMsgValidGWZoneFR1_flg/1 -> [VINP_CANMsgValidGWZoneFR1_flg]
  [VINP_CANMsgValidGWZoneFR1_flg] -> AntiTheft/17(VINP_CANMsgValidGWZoneFR1_flg)
  [VINP_CANMsgValidGWZoneDR1_flg] -> AntiTheft/16(VINP_CANMsgValidGWZoneDR1_flg)
  RoomLamp/1(VBCM_RoomLampH_flg) -> [VBCM_RoomLampH_flg]
  RoomLamp/2(VBCM_RoomLampL_flg) -> VBCM_RoomLampL_flg/1
  [task_time_s] -> RoomLamp/1(task_time_s)
  [VINP_DrDoorSW_flg] -> RoomLamp/6(VINP_DrDoorSW_flg)
  [VINP_PsDoorSW_flg] -> RoomLamp/7(VINP_PsDoorSW_flg)
  [VINP_RLDoorSW_flg] -> RoomLamp/8(VINP_RLDoorSW_flg)
  [VINP_RRDoorSW_flg] -> RoomLamp/9(VINP_RRDoorSW_flg)
  Constant18/1 -> RoomLamp/15(KBCM_RmLpKeyInT_s)  "2400"
  VDKC_PDKeyAreaLockUnlock_enum/1 -> RoomLamp/13(VINP_PDKeyAreaLockUnlock_enum)
  Constant19/1 -> RoomLamp/16(KBCM_RmLpKeyMissT_s)  "600"
  VDKC_PDKeyAreaPS_enum/1 -> RoomLamp/14(VINP_PDKeyAreaPS_enum)
  VINP_DiagFLTC_mA/1 -> [VINP_DiagFLTC_mA]
  VINP_DiagFRTC_mA/1 -> [VINP_DiagFRTC_mA]
  VINP_DiagRLTC_mA/1 -> [VINP_DiagRLTC_mA]
  VINP_DiagRRTC_mA/1 -> [VINP_DiagRRTC_mA]
  VINP_DiagDRLOFF_flg/1 -> [VINP_DiagDRLOFF_flg]
  VINP_DiagFMHT_s/1 -> [VINP_DiagFMHT_s]
  [task_time_s] -> ExteriorLight/1(task_time_s)
  FlasherSignal/4(VBCM_OutMode_enum) -> [VBCM_OutMode_enum]
  FlasherSignal/5(VBCM_BCMBuzzerReq_flg) -> VBCM_BCMBuzzerReq_flg/1
  FlasherSignal/6(VBCM_DiagFLTS_flg) -> VBCM_DiagFLTS_flg/1
  FlasherSignal/7(VBCM_DiagFRTS_flg) -> VBCM_DiagFRTS_flg/1
  FlasherSignal/8(VBCM_DiagRLTS_flg) -> VBCM_DiagRLTS_flg/1
  FlasherSignal/9(VBCM_DiagRRTS_flg) -> VBCM_DiagRRTS_flg/1
  [task_time_s] -> FlasherSignal/22(task_time_s)
  VINP_SRRBSDWarnL_enum/1 -> [VINP_SRRBSDWarnL_enum]
  VINP_IVILockSoundSWSta_flg/1 -> AntiTheft/19(VINP_IVILockSoundSWSta_flg)
  AntiTheft/17(VBCM_LockAlarm_enum) -> VBCM_LockAlarm_enum/1
  CenterDoorLock/10(VBCM_fUnlockSingle_flg) -> VBCM_fUnlockSingle_flg/1
  VINP_FlashfUnlockSingle_flg/1 -> CenterDoorLock/17(VINP_FlashfUnlockSingle_flg)
  [VINP_SRRODAWarnR_enum] -> ExteriorLight/13(VINP_SRRODAWarnR_enum)
  [VINP_SRRODAWarnL_enum] -> ExteriorLight/14(VINP_SRRODAWarnL_enum)
  [VINP_SRRBSDWarnL_enum] -> ExteriorLight/16(VINP_SRRBSDWarnL_enum)
  [VINP_SRRBSDWarnR_enum] -> ExteriorLight/15(VINP_SRRBSDWarnR_enum)
  VINP_AmbLightSW_flg/1 -> Personal_Setting/4(VINP_AmbLightSW_flg)
  VINP_AmbLightWlcmLightSW_flg/1 -> Personal_Setting/6(VINP_AmbLightWlcmLightSW_flg)
  VINP_AmbLightDimInDarkSW_flg/1 -> Personal_Setting/8(VINP_AmbLightDimInDarkSW_flg)
  VINP_LINKtoDRIVE_flg/1 -> Personal_Setting/10(VINP_LINKtoDRIVE_flg)
  VINP_AmbLighLowBatAlertSW_flg/1 -> Personal_Setting/12(VINP_AmbLighLowBatAlertSW_flg)
  VINP_AmbLighSafetyAlertSW_flg/1 -> Personal_Setting/14(VINP_AmbLighSafetyAlertSW_flg)
  VINP_AmbLightBrightnessSet_enum/1 -> Personal_Setting/23(VINP_AmbLightBrightnessSet_enum)
  VINP_AmbLightColorSet_enum/1 -> Personal_Setting/16(VINP_AmbLightColorSet_enum)
  VINP_FlashAmbColorSta5_enum/1 -> Personal_Setting/21(VINP_FlashAmbColorSta5_enum)
  VINP_FlashAmbColorSta7_enum/1 -> Personal_Setting/22(VINP_FlashAmbColorSta7_enum)
  VINP_FlashAmbBrightnessSta5_enum/1 -> Personal_Setting/28(VINP_FlashAmbBrightnessSta5_enum)
  VINP_FlashAmbBrightnessSta7_enum/1 -> Personal_Setting/29(VINP_FlashAmbBrightnessSta7_enum)
  VINP_FlashAmbColorSta1_enum/1 -> Personal_Setting/17(VINP_FlashAmbColorSta1_enum)
  VINP_FlashAmbColorSta2_enum/1 -> Personal_Setting/18(VINP_FlashAmbColorSta2_enum)
  VINP_FlashAmbColorSta3_enum/1 -> Personal_Setting/19(VINP_FlashAmbColorSta3_enum)
  VINP_FlashAmbColorSta4_enum/1 -> Personal_Setting/20(VINP_FlashAmbColorSta4_enum)
  VINP_FlashAmbBrightnessSta1_enum/1 -> Personal_Setting/24(VINP_FlashAmbBrightnessSta1_enum)
  VINP_FlashAmbBrightnessSta2_enum/1 -> Personal_Setting/25(VINP_FlashAmbBrightnessSta2_enum)
  VINP_FlashAmbBrightnessSta3_enum/1 -> Personal_Setting/26(VINP_FlashAmbBrightnessSta3_enum)
  VINP_FlashAmbBrightnessSta4_enum/1 -> Personal_Setting/27(VINP_FlashAmbBrightnessSta4_enum)
  VINP_FlashAmbDimEN_enum/1 -> Personal_Setting/9(VINP_FlashAmbDimEN_enum)
  VINP_FlashAmbLinkDriSta_enum/1 -> Personal_Setting/11(VINP_FlashAmbLinkDriSta_enum)
  VINP_FlashAmbPwrWarnEN_enum/1 -> Personal_Setting/13(VINP_FlashAmbPwrWarnEN_enum)
  VINP_FlashAmbODAEN_enum/1 -> Personal_Setting/15(VINP_FlashAmbODAEN_enum)
  VINP_FlashAmbFunEN_enum/1 -> Personal_Setting/5(VINP_FlashAmbFunEN_enum)
  VINP_FlashAmbWelEN_enum/1 -> Personal_Setting/7(VINP_FlashAmbWelEN_enum)
  VINP_UserSet_enum/1 -> Personal_Setting/2(UserNow)
  VINP_CANMsgValidIVI1_flg/1 -> [VINP_CANMsgValidIVI1_flg]
  [VINP_CANMsgValidIVI1_flg] -> AntiTheft/18(VINP_CANMsgValidIVI1_flg)
  [VINP_CANMsgValidIVI1_flg] -> Personal_Setting/3(VINP_CANMsgValidIVI1_flg)
  Personal_Setting/22(FDC_BCM_AmbBrightSta_Sta) -> [FDC_BCM_AmbBrightSta_Sta]  "VBCM_AmbBrightSta_enum"
  Personal_Setting/15(FDC_BCM_AmbColorSta_Sta) -> [FDC_BCM_AmbColorSta_Sta]  "VBCM_AmbColorSta_enum"
  Personal_Setting/11(FDC_BCM_AmbPwrWarnEN_Sta) -> [FDC_BCM_AmbPwrWarnEN_Sta]  "VBCM_AmbPwrWarnEN_flg"
  Personal_Setting/13(FDC_BCM_AmbODAEN_Sta) -> [FDC_BCM_AmbODAEN_Sta]  "VBCM_AmbODAEN_flg"
  Personal_Setting/9(FDC_BCM_AmbLinkDriSta_Sta) -> [FDC_BCM_AmbLinkDriSta_Sta]  "VBCM_AmbLinkDriSta_flg"
  Personal_Setting/2(VBCM_UserNow_enum) -> VBCM_UserNow_enum/1  "VBCM_UserNow_enum"
  Personal_Setting/23(VBCM_AmbBrightnessSta1_enum) -> VBCM_AmbBrightnessSta1_enum/1  "VBCM_AmbBrightnessSta1_enum"
  Personal_Setting/7(FDC_BCM_AmbDimEN_Sta) -> [FDC_BCM_AmbDimEN_Sta]  "VBCM_AmbDimEN_flg"
  Personal_Setting/24(VBCM_AmbBrightnessSta2_enum) -> VBCM_AmbBrightnessSta2_enum/1  "VBCM_AmbBrightnessSta2_enum"
  Personal_Setting/21(VBCM_AmbColorSta7_enum) -> VBCM_AmbColorSta7_enum/1  "VBCM_AmbColorSta7_enum"
  Personal_Setting/25(VBCM_AmbBrightnessSta3_enum) -> VBCM_AmbBrightnessSta3_enum/1  "VBCM_AmbBrightnessSta3_enum"
  Personal_Setting/5(FDC_BCM_AmbWelEN_Sta) -> [FDC_BCM_AmbWelEN_Sta]  "VBCM_AmbWelEN_flg"
  Personal_Setting/20(VBCM_AmbColorSta5_enum) -> VBCM_AmbColorSta5_enum/1  "VBCM_AmbColorSta5_enum"
  Personal_Setting/26(VBCM_AmbBrightnessSta4_enum) -> VBCM_AmbBrightnessSta4_enum/1  "VBCM_AmbBrightnessSta4_enum"
  Personal_Setting/19(VBCM_AmbColorSta4_enum) -> VBCM_AmbColorSta4_enum/1  "VBCM_AmbColorSta4_enum"
  Personal_Setting/27(VBCM_AmbBrightnessSta5_enum) -> VBCM_AmbBrightnessSta5_enum/1  "VBCM_AmbBrightnessSta5_enum"
  Personal_Setting/3(FDC_BCM_AmbFunEN_Sta) -> [FDC_BCM_AmbFunEN_Sta]  "VBCM_AmbFunEN_flg"
  Personal_Setting/18(VBCM_AmbColorSta3_enum) -> VBCM_AmbColorSta3_enum/1  "VBCM_AmbColorSta3_enum"
  Personal_Setting/28(VBCM_AmbBrightnessSta7_enum) -> VBCM_AmbBrightnessSta7_enum/1  "VBCM_AmbBrightnessSta7_enum"
  Personal_Setting/17(VBCM_AmbColorSta2_enum) -> VBCM_AmbColorSta2_enum/1  "VBCM_AmbColorSta2_enum"
  Personal_Setting/16(VBCM_AmbColorSta1_enum) -> VBCM_AmbColorSta1_enum/1  "VBCM_AmbColorSta1_enum"
  Personal_Setting/14(VBCM_AmbODAENMem_enum) -> VBCM_AmbODAENFlash_enum/1  "VBCM_AmbODAENFlash_enum"
  Personal_Setting/12(VBCM_AmbPwrWarnENMem_enum) -> VBCM_AmbPwrWarnENFlash_enum/1  "VBCM_AmbPwrWarnENFlash_enum"
  Personal_Setting/10(VBCM_AmbLinkDriStaMem_enum) -> VBCM_AmbLinkDriStaFlash_enum/1  "VBCM_AmbLinkDriStaFlash_enum"
  Personal_Setting/8(VBCM_AmbDimENMem_enum) -> VBCM_AmbDimENFlash_enum/1  "VBCM_AmbDimENFlash_enum"
  Personal_Setting/6(VBCM_AmbWelENMem_enum) -> VBCM_AmbWelENFlash_enum/1  "VBCM_AmbWelENFlash_enum"
  Personal_Setting/4(VBCM_AmbFunENMem_enum) -> VBCM_AmbFunENFlash_enum/1  "VBCM_AmbFunENFlash_enum"
  FlasherSignal/10(VBCM_HazardIND_flg) -> VBCM_HazardIND_flg/1
  VINP_SASAngle_Deg/1 -> CSW/12(VINP_SASAngle_deg)
  VINP_CSW2FWasSwSta_enum/1 -> CSW/11(VINP_CSW2FWasSwSta_enum)
  VINP_CSW2FWipSwSta_enum/1 -> CSW/9(VINP_CSW2FWipSwSta_enum)
  VINP_CSW2RWipWasSwSta_enum/1 -> CSW/15(VINP_CSW2RWIPWasSwSta_enum)
  VINP_CSW2DimSwSta_flg/1 -> CSW/3(VINP_CSW2DimSwSta_flg)
  VINP_CSW2PassSWSta_flg/1 -> CSW/5(VINP_CSW2PassSWSta_flg)
  VUNP_CSW2TurnSwSta_enum/1 -> CSW/7(VINP_CSW2TurnSwSta_enum)
  [task_time_s] -> CSW/1(task_time_s)
  Unit Delay2/1 -> CSW/14(VINP_LBeam_flg)
  [VBCM_LBeam_flg] -> Unit Delay2/1
  VINP_CSWTurnSWSta_enum/1 -> [VINP_CSWTurnSWSta_enum]
  [VINP_CSWTurnSWSta_enum] -> CSW/6(VINP_CSWTurnSwSta_enum)
  VINP_CSWDimSw_flg/1 -> [VINP_CSWDimSw_flg]
  VINP_CSWPassSWSta_flg/1 -> [VINP_CSWPassSWSta_flg]
  [VINP_CSWDimSw_flg] -> CSW/2(VINP_CSWDimSwSta_flg)
  [VINP_CSWPassSWSta_flg] -> CSW/4(VINP_CSWPassSWSta_flg)
  VINP_CSWFWasSWSta_enum/1 -> [VINP_CSWFWasSWSta_enum]
  VINP_CSWRWasSWSta_enum/1 -> [VINP_CSWRWasSWSta_enum]
  VINP_CSWRWipIntSwSta_enum/1 -> [VINP_CSWRWipIntSwSta_enum]
  VINP_CSWFWipSWSta_enum/1 -> [VINP_CSWFWipSWSta_enum]
  [VINP_CSWFWipSWSta_enum] -> CSW/8(VINP_CSWFWipSwSta_enum)
  [VINP_CSWFWasSWSta_enum] -> CSW/10(VINP_CSWFWasSwSta_enum)
  [VINP_CSWRWipIntSwSta_enum] -> CSW/16(VINP_CSWRWipIntSwSta_enum)
  [VINP_CSWRWasSWSta_enum] -> CSW/17(VINP_CSWRWasSWSta_enum)
  CSW/4(VBCM_FWipSwSta_enum) -> [VBCM_FWipSwSta_enum]
  CSW/5(VBCM_FWasSwSta_enum) -> [VBCM_FWasSwSta_enum]
  CSW/6(VBCM_RWasSwSta_enum) -> [VBCM_RWasSwSta_enum]
  CSW/1(VBCM_DimSwSta_flg) -> [VBCM_DimSwSta_flg]
  CSW/2(VBCM_PassSWSta_flg) -> [VBCM_PassSWSta_flg]
  CSW/3(VBCM_TurnSwSta_enum) -> [VBCM_TurnSwSta_enum]
  CSW/7(VBCM_RWipIntSwSta_enum) -> [VBCM_RWipIntSwSta_enum]
  [VBCM_FWasSwSta_enum] -> WasherWiper/2(VINP_CSWFWasSWSta_enum)
  [VBCM_RWipIntSwSta_enum] -> WasherWiper/6(VINP_CSWRWipIntSwSta_enum)
  [VBCM_FWipSwSta_enum] -> WasherWiper/3(VINP_CSWFWipSWSta_enum)
  [VBCM_RWasSwSta_enum] -> WasherWiper/8(VINP_CSWRWasSWSta_enum)
  [VBCM_TurnSwSta_enum] -> FlasherSignal/5(VINP_CSWTurnSWSta_enum)
  [VBCM_PassSWSta_flg] -> ExteriorLight/7(VINP_CSWPassSWSta_flg)
  [VBCM_DimSwSta_flg] -> ExteriorLight/6(VINP_CSWDimSw_flg)
  VINP_CANMsgValidShifter2_flg/1 -> CSW/18(VINP_CANMsgValidShifter2_flg)
  Personal_Setting/29(VBCM_SPTGENFun_flg) -> [VBCM_SPTGENFun_flg]  "VBCM_SPTGENFun_flg"
  VINP_IVIPTGUSStaSW_flg/1 -> Personal_Setting/30(VINP_IVIPTGUSStaSW_flg)
  Personal_Setting/30(VBCM_SPTGENFunMem_enum) -> VBCM_SPTGENFunMem_enum/1  "VBCM_SPTGENFunMem_enum"
  VINP_FlashIVIPTGUSStaSW_enum/1 -> Personal_Setting/31(VINP_FlashSPTGENFun_enum)
  Personal_Setting/31(VBCM_TurnSwTSetSta_enum) -> [VBCM_TurnSwTSetSta_enum]  "VBCM_TurnSwTSetSta_enum"
  Personal_Setting/32(VBCM_TurnSwTimeSetSta123_enum) -> VBCM_TurnSwTimeSetSta123_enum/1  "VBCM_TurnSwTimeSetSta123_enum"
  Personal_Setting/33(VBCM_TurnSwTimeSetSta457_enum) -> VBCM_TurnSwTimeSetSta457_enum/1  "VBCM_TurnSwTimeSetSta457_enum"
  VINP_TurnSwTimeSet_enum/1 -> Personal_Setting/32(VINP_TurnSwTimeSet_enum)
  VINP_FlashTurnSwTimeSetSta123_enum/1 -> Personal_Setting/33(VINP_FlashTurnSwTimeSetSta123_enum)
  VINP_FlashTurnSwTimeSetSta457_enum/1 -> Personal_Setting/34(VINP_FlashTurnSwTimeSetSta457_enum)
  [VBCM_TurnSwTSetSta_enum] -> CSW/13(VINP_TurnSwTimeSet_enum)
  [VINP_CANMsgValidIVI2_flg] -> Personal_Setting/35(VINP_CANMsgValidIVI2_flg)
  VTPM_TPMSTLCmd_flg/1 -> FlasherSignal/23(VTPM_TPMSTLCmd_flg)
  [VINP_DrDoorSW_flg] -> CenterDoorLock/18(VINP_DrDoorSW_flg)
  [VINP_PsDoorSW_flg] -> CenterDoorLock/19(VINP_PsDoorSW_flg)
  [VINP_RLDoorSW_flg] -> CenterDoorLock/20(VINP_RLDoorSW_flg)
  [VINP_RRDoorSW_flg] -> CenterDoorLock/21(VINP_RRDoorSW_flg)
  Constant6/1 -> CenterDoorLock/26(KBCM_CmdKeepT_s)
  Constant7/1 -> CenterDoorLock/27(KBCM_HandleLampKeepT_s)
  VINP_FLHandleClose_flg/1 -> CenterDoorLock/22(VINP_FLHandleClose_flg)
  VINP_FRHandleClose_flg/1 -> CenterDoorLock/23(VINP_FRHandleClose_flg)
  VINP_RLHandleClose_flg/1 -> CenterDoorLock/24(VINP_RLHandleClose_flg)
  VINP_RRHandleClose_flg/1 -> CenterDoorLock/25(VINP_RRHandleClose_flg)
  CenterDoorLock/11(VBCM_FDLHandleLampCmd_flg) -> VBCM_FDLHandleLampCmd_flg/1
  CenterDoorLock/12(VBCM_FDRHandleLampCmd_flg) -> VBCM_FDRHandleLampCmd_flg/1
  CenterDoorLock/13(VBCM_FDHandleCmd_enum) -> VBCM_FDHandleCmd_enum/1
  ExteriorLight/13(VBCM_HBeamADB_flg) -> VBCM_HBeamADB_flg/1
  [FDC_BCM_AmbPwrWarnEN_Sta] -> Amb/16(VINP_AmbPwrWarnEN_flg)
  [FDC_BCM_AmbLinkDriSta_Sta] -> Amb/19(VINP_AmbLinkDriSta_flg)
  [FDC_BCM_AmbBrightSta_Sta] -> Amb/17(VINP_AmbBrightnessSta_enum)
  [FDC_BCM_AmbColorSta_Sta] -> Amb/18(VINP_AmbColorSta_enum)
  [VINP_SRRODASoundL_flg] -> Amb/8(VINP_SRRODASoundL_flg)
  [VINP_SRRODASoundR_flg] -> Amb/9(VINP_SRRODASoundR_flg)
  [VINP_SRRBSDWarnL_enum] -> Amb/10(VINP_SRRBSDWarnL_enum)
  [VINP_SRRBSDWarnR_enum] -> Amb/11(VINP_SRRBSDWarnR_enum)
  [FDC_BCM_AmbODAEN_Sta] -> Amb/15(VINP_AmbODAEN_flg)
  [VBCM_FlashAntitheft_enum] -> Amb/21(EEP_AntitheftSta)
  [FDC_BCM_AmbFunEN_Sta] -> Amb/12(VINP_AmbFunEN_flg)
  [FDC_BCM_AmbWelEN_Sta] -> Amb/13(VINP_AmbWelEN_flg)
  [FDC_BCM_AmbDimEN_Sta] -> Amb/14(VINP_AmbDimEN_flg)
  [VINP_IVINightModeSta_flg] -> Amb/3(VINP_IVINightModeSta_flg)
  [VBCM_AllDoorSW_flg] -> Amb/4(VBCM_AllDoorSW_flg)
  [VPMM_PwrSta_enum] -> Amb/5(VPMM_PwrSta_enum)
  [VBCM_PosLamp_flg] -> Amb/6(VBCM_PosLamp_flg)
  [VBCM_WakeUp_flg] -> Amb/7(VBCM_WakeUp_flg)
  [VBCM_AntitheftSta_enum] -> Amb/20(AntitheftSta)
  [task_time_s] -> Amb/1(task_time_s)
  VINP_IVIPWModeReq_enum/1 -> Amb/2(VINP_IVIPWModeReq_enum)
  VINP_HVBattSOCDis_pct/1 -> Amb/22(VINP_HVBattSOCDis_pct)
  Amb/1(VBCM_LampPwr_flg) -> VBCM_LampPwr_flg/1
  Amb/2(VBCM_AmbLightBreath1_enum) -> VBCM_AmbLightBreath1_enum/1  "VBCM_AmbLightBreath1_enum"
  Amb/3(VBCM_AmbLightBreath2_enum) -> VBCM_AmbLightBreath2_enum/1  "VBCM_AmbLightBreath2_enum"
  Amb/4(VBCM_AmbLightBreath3_enum) -> VBCM_AmbLightBreath3_enum/1  "VBCM_AmbLightBreath3_enum"
  Amb/5(VBCM_AmbLightBreath4_enum) -> VBCM_AmbLightBreath4_enum/1  "VBCM_AmbLightBreath4_enum"
  Amb/6(VBCM_AmbLightBreath5_enum) -> VBCM_AmbLightBreath5_enum/1  "VBCM_AmbLightBreath5_enum"
  Amb/7(VBCM_AmbLightBreath6_enum) -> VBCM_AmbLightBreath6_enum/1  "VBCM_AmbLightBreath6_enum"
  Amb/8(VBCM_AmbLightBrightness1_enum) -> VBCM_AmbLightBrightness1_enum/1  "VBCM_AmbLightBrightness1_enum"
  Amb/9(VBCM_AmbLightBrightness2_enum) -> VBCM_AmbLightBrightness2_enum/1  "VBCM_AmbLightBrightness2_enum"
  Amb/10(VBCM_AmbLightBrightness3_enum) -> VBCM_AmbLightBrightness3_enum/1  "VBCM_AmbLightBrightness3_enum"
  Amb/11(VBCM_AmbLightBrightness4_enum) -> VBCM_AmbLightBrightness4_enum/1  "VBCM_AmbLightBrightness4_enum"
  Amb/12(VBCM_AmbLightBrightness5_enum) -> VBCM_AmbLightBrightness5_enum/1  "VBCM_AmbLightBrightness5_enum"
  Amb/13(VBCM_AmbLightBrightness6_enum) -> VBCM_AmbLightBrightness6_enum/1  "VBCM_AmbLightBrightness6_enum"
  Amb/14(VBCM_AmbLightColor1_enum) -> VBCM_AmbLightColor1_enum/1  "VBCM_AmbLightColor1_enum"
  Amb/15(VBCM_AmbLightColor2_enum) -> VBCM_AmbLightColor2_enum/1  "VBCM_AmbLightColor2_enum"
  Amb/16(VBCM_AmbLightColor3_enum) -> VBCM_AmbLightColor3_enum/1  "VBCM_AmbLightColor3_enum"
  Amb/17(VBCM_AmbLightColor4_enum) -> VBCM_AmbLightColor4_enum/1  "VBCM_AmbLightColor4_enum"
  Amb/18(VBCM_AmbLightColor5_enum) -> VBCM_AmbLightColor5_enum/1  "VBCM_AmbLightColor5_enum"
  Amb/19(VBCM_AmbLightColor6_enum) -> VBCM_AmbLightColor6_enum/1  "VBCM_AmbLightColor6_enum"
  VTHC_Z1UP_flg/1 -> Amb/23(VTHC_Z1UP_flg)
  VTHC_Z2UP_flg/1 -> Amb/24(VTHC_Z2UP_flg)
  VTHC_Z1DN_flg/1 -> Amb/25(VTHC_Z1DN_flg)
  VTHC_Z2DN_flg/1 -> Amb/26(VTHC_Z2DN_flg)
  [task_time_s] -> CenterDoorLock/1(task_time_s)
  VINP_ApproachUnlockSW_flg/1 -> Personal_Setting/36(VINP_ApproachUnlockSW_flg)
  VINP_FlashWalkInUnLkEN_enum/1 -> Personal_Setting/37(VINP_FlashWalkInUnLkEn_enum)
  VINP_WalkawayLockSW_flg/1 -> Personal_Setting/38(VINP_WalkawayLockSW_flg)
  VINP_FlashWalkOutLkEN_enum/1 -> Personal_Setting/39(VINP_FlashWalkOutLkEn_enum)
  VINP_RoomLampMode_flg/1 -> Personal_Setting/40(VINP_RoomLampMode_flg)
  VINP_FlashRmLpModeEN_enum/1 -> Personal_Setting/41(VINP_FlashRmLpModeEN_enum)
  VINP_SetUnlockSingle_flg/1 -> Personal_Setting/42(VINP_SetUnlockSingle_flg)
  VINP_FlashLockSettingSta_enum/1 -> Personal_Setting/43(VINP_FlashLockSettingSta_enum)
  VINP_FollowMeSW_flg/1 -> Personal_Setting/44(VINP_FollowMeSW_flg)
  VINP_FlashFollowMeENFun_enum/1 -> Personal_Setting/45(VINP_FlashFollowMeENFun_enum)
  Personal_Setting/34(FDC_BCM_WalkInUnLkEnFun_Sta) -> [FDC_BCM_WalkInUnLkEnFun_Sta]  "VBCM_WalkInUnLkENFunSta_flg"
  Personal_Setting/35(VBCM_WalkInUnLkEnMem_enum) -> VBCM_WalkInUnLkENMem_enum/1  "VBCM_WalkInUnLkENMem_enum"
  Personal_Setting/37(VBCM_WalkOutLkEnMem_enum) -> VBCM_WalkOutLkENMem_enum/1  "VBCM_WalkOutLkENMem_enum"
  Personal_Setting/39(VBCM_RmLpModeENMem_enum) -> VBCM_RmLpModeENMem_enum/1  "VBCM_RmLpModeENMem_enum"
  Personal_Setting/41(VBCM_LockSettingStaMem_enum) -> VBCM_LockSettingStaMem_enum/1  "VBCM_LockSettingStaMem_enum"
  Personal_Setting/43(VBCM_FollowMeENMem_enum) -> VBCM_FollowMeENMem_enum/1  "VBCM_FollowMeENMem_enum"
  Personal_Setting/36(FDC_BCM_WalkOutLkEnFun_Sta) -> [FDC_BCM_WalkOutLkEnFun_Sta]  "VBCM_WalkOutLkENFunSta_flg"
  Personal_Setting/38(FDC_BCM_RmLpModeENFun_Sta) -> [FDC_BCM_RmLpModeENFun_Sta]  "VBCM_RmLpModeENFunSta_flg"
  Personal_Setting/40(VBCM_LockSetting_flg) -> [VBCM_LockSetting_flg]  "VBCM_LockSetting_flg"
  Personal_Setting/42(FDC_BCM_FollowMeENFun_Sta) -> [FDC_BCM_FollowMeENFun_Sta]  "VBCM_FollowMeENFunSta_flg"
  [FDC_BCM_WalkInUnLkEnFun_Sta] -> AntiTheft/20(FDC_BCM_WalkInUnLkEnFun_Sta)
  [FDC_BCM_WalkOutLkEnFun_Sta] -> AntiTheft/21(FDC_BCM_WalkOutLkEnFun_Sta)
  Personal_Setting/1(Loadbar) -> [Loadbar]
  [Loadbar] -> AntiTheft/22(Loadbar)
  [FDC_BCM_RmLpModeENFun_Sta] -> RoomLamp/10(FDC_BCM_RmLpModeENFun_Sta)
  [VBCM_LockSetting_flg] -> CenterDoorLock/2(VBCM_LockSetting_flg)
  [FDC_BCM_FollowMeENFun_Sta] -> ExteriorLight/23(FDC_BCM_FollowMeENFun_Sta)
  AntiTheft/18(VBCM_HoodRelCmd_flg) -> VBCM_HoodRelCmd_flg/1
  VINP_IVIFrTrunkUnlockReqSta_flg/1 -> Detect Increase/1
  [VTQD_ShiftGearPosn_enum] -> AntiTheft/24(VINP_ShiftGearPosn_enum)
  Amb/20(VBCM_LampPwrReady_flg) -> Terminator7/1
  VINP_FLTurnLPErr_flg/1 -> FlasherSignal/26(VINP_FLTurnLPErr_flg)
  VINP_FRTurnLPErr_flg/1 -> FlasherSignal/27(VINP_FRTurnLPErr_flg)
  VINP_RLTurnLPErr_flg/1 -> FlasherSignal/28(VINP_RLTurnLPErr_flg)
  VINP_RRTurnLPErr_flg/1 -> FlasherSignal/29(VINP_RRTurnLPErr_flg)
  VINP_HRLTurnLPNormalSta_flg/1 -> FlasherSignal/30(VINP_HRLTurnLPNormalSta_flg)
  VINP_HRRTurnLPHNormalSta_flg/1 -> FlasherSignal/31(VINP_HRRTurnLPHNormalSta_flg)
  FlasherSignal/11(VBCM_WelcomeLight_enum) -> VBCM_WelcomeLight_enum/1
  Detect Increase/1 -> AntiTheft/23(VBCM_IVIFrTrunkUnlockReqRising_flg)
  [VBCM_FlashAntitheft_enum] -> AntiTheft/13(VBCM_FlashAntitheft_enum)
  [VINP_CANMsgValidGWZoneFR1_flg] -> FlasherSignal/24(VINP_CANMsgValidZONEFR1_flg)
  [VINP_CANMsgValidGWZoneDR1_flg] -> FlasherSignal/25(VINP_CANMsgValidZONEDR1_flg)
  VINP_ZRPTGRDILCmd_enum/1 -> FlasherSignal/33(VINP_ZRPTGRDILCmd_enum)
  VINP_CANMsgValidZONER1_flg/1 -> FlasherSignal/32(VINP_CANMsgValidZONER1_flg)
  VINP_IVIPTGOpenHeight_enum/1 -> Personal_Setting/46(VINP_IVIPTGOpenHeight_enum)
  VINP_BPPTGIsSetHeightSta_flg/1 -> Personal_Setting/51(VINP_BPPTGIsSetHeightSta_flg)
  VINP_FlashPTGUserHeight7_cnt/1 -> Personal_Setting/58(VINP_FlashPTGUserHeight7_cnt)
  VINP_PTGLeftHallPosn_cnt/1 -> Personal_Setting/52(VINP_PTGLeftHallPosn_cnt)
  VINP_FlashPTGUserHeight1_cnt/1 -> Personal_Setting/53(VINP_FlashPTGUserHeight1_cnt)
  VINP_FlashPTGUserHeight2_cnt/1 -> Personal_Setting/54(VINP_FlashPTGUserHeight2_cnt)
  VINP_FlashPTGUserHeight3_cnt/1 -> Personal_Setting/55(VINP_FlashPTGUserHeight3_cnt)
  VINP_FlashPTGUserHeight4_cnt/1 -> Personal_Setting/56(VINP_FlashPTGUserHeight4_cnt)
  VINP_FlashPTGUserHeight5_cnt/1 -> Personal_Setting/57(VINP_FlashPTGUserHeight5_cnt)
  Personal_Setting/44(VBCM_PTGOpenHeightSta_enum) -> VBCM_PTGOpenHeightSta_enum/1  "VBCM_PTGOpenHeightSta_enum"
  Personal_Setting/45(VBCM_UserHeightSet_cnt) -> VBCM_UserHeightSet_cnt/1  "VBCM_UserHeightSet_cnt"
  Personal_Setting/46(VBCM_PTGUserHeight1_cnt) -> VBCM_PTGUserHeight1_cnt/1  "VBCM_PTGUserHeight1_cnt"
  Personal_Setting/47(VBCM_PTGUserHeight2_cnt) -> VBCM_PTGUserHeight2_cnt/1  "VBCM_PTGUserHeight2_cnt"
  Personal_Setting/48(VBCM_PTGUserHeight3_cnt) -> VBCM_PTGUserHeight3_cnt/1  "VBCM_PTGUserHeight3_cnt"
  Personal_Setting/49(VBCM_PTGUserHeight4_cnt) -> VBCM_PTGUserHeight4_cnt/1  "VBCM_PTGUserHeight4_cnt"
  Personal_Setting/50(VBCM_PTGUserHeight5_cnt) -> VBCM_PTGUserHeight5_cnt/1  "VBCM_PTGUserHeight5_cnt"
  Personal_Setting/51(VBCM_PTGUserHeight7_cnt) -> VBCM_PTGUserHeight7_cnt/1  "VBCM_PTGUserHeight7_cnt"
  VINP_FlashPTGOpenHeight12_enum/1 -> Personal_Setting/47(VINP_FlashPTGOpenHeight12_enum)
  VINP_FlashPTGOpenHeight34_enum/1 -> Personal_Setting/48(VINP_FlashPTGOpenHeight34_enum)
  VINP_FlashPTGOpenHeight57_enum/1 -> Personal_Setting/49(VINP_FlashPTGOpenHeight57_enum)
  Personal_Setting/52(VBCM_PTGOpenHeight12_enum) -> VBCM_PTGOpenHeight12_enum/1  "VBCM_PTGOpenHeight12_enum"
  Personal_Setting/53(VBCM_PTGOpenHeight34_enum) -> VBCM_PTGOpenHeight34_enum/1  "VBCM_PTGOpenHeight34_enum"
  Personal_Setting/54(VBCM_PTGOpenHeight57_enum) -> VBCM_PTGOpenHeight57_enum/1  "VBCM_PTGOpenHeight57_enum"
  [VINP_TailgateSW_flg] -> PTG/4(VINP_TailgateSW_flg)
  [VDKC_PCommandToBCM_enum] -> PTG/7(VINP_PCommandToBCM_enum)
  [VPMM_PwrSta_enum] -> PTG/8(VPMM_PwrSta_eunm)
  [VTQD_ShiftGearPosn_enum] -> PTG/9(VTQD_ShiftGearPosn_enum)
  [VINP_VehSpeed_kph] -> PTG/11(VINP_VehSpeed_kph)
  [VBCM_SPTGENFun_flg] -> PTG/10(VBCM_SPTGENFun_flg)
  Constant10/1 -> PTG/12(KBCM_DelayTSW_flg)
  Constant11/1 -> PTG/13(KBCM_ReDetectT_K)
  Constant12/1 -> PTG/14(KBCM_SPTGDetectT_sec)
  Constant13/1 -> PTG/15(KBCM_SPTGLeave_flg)
  Constant15/1 -> PTG/16(KBCM_SPTGWaitDKC_sec)
  VDKC_PDKeyAreaPTG_enum/1 -> PTG/2(VINP_PDKeyAreaPTG_enum)
  VDKC_KeyAreaSPTGSta_enum/1 -> PTG/3(VDKC_KeyAreaSPTGSta_enum)
  VAPM_PASDRMR_cm/1 -> PTG/5(VAPM_PASDRMR_cm)
  VAPM_PASDRML_cm/1 -> PTG/6(VAPM_PASDRML_cm)
  PTG/1(VBCM_SPTGDet_flg) -> [VBCM_SPTGDet_flg]  "VBCM_SPTGDet_flg"
  PTG/2(VBCM_APSOpenPTG_flg) -> [VBCM_APSOpenPTG_flg]  "VBCM_APSOpenPTG_flg"
  VINP_CANMsgValidDKC1_flg/1 -> Terminator8/1
  [task_time_s] -> Personal_Setting/1(task_time_s)
  VINP_DrSeatSta_enum/1 -> AntiTheft/25(VINP_DrSeatSta_enum)
  VINP_RAPSBCMLockReqCmd_flg/1 -> AntiTheft/26(VINP_RAPSBCMLockReqCmd_flg)
  [VINP_RAPSErrWarn_enum] -> AntiTheft/27(VINP_RAPSErrWarn_enum)
  VINP_RAPSErrWarn_enum/1 -> [VINP_RAPSErrWarn_enum]
  [VTQD_ShiftGearPosn_enum] -> CenterDoorLock/28(VTQD_ShiftGearPosn_enum)
  [VBCM_AutoUnlockSta_flg] -> CenterDoorLock/30(VBCM_AutoUnlockSta_flg)
  [VBCM_AutoLockSta_flg] -> CenterDoorLock/29(VBCM_AutoLockSta_flg)
  [VDKC_PDKeyAreaRAPSSta_enum] -> FlasherSignal/36(VDKC_PDKeyAreaRAPSSta_enum)
  [VINP_RAPSBCMLamp_enum] -> FlasherSignal/34(VINP_RAPSBCMLamp_enum)
  [VINP_APSStaSystem_enum] -> FlasherSignal/35(VINP_APSStaSystem_enum)
  [VINP_RAPSErrWarn_enum] -> FlasherSignal/37(VINP_RAPSErrWarn_enum)
  [VINP_APSStaSystem_enum] -> PowerMirror/8(VINP_APSStaSystem_enum)
  VINP_RAPSBCMLamp_enum/1 -> [VINP_RAPSBCMLamp_enum]
  VINP_APSStaSystem_enum/1 -> [VINP_APSStaSystem_enum]
  VDKC_PDKeyAreaRAPSSta_enum/1 -> [VDKC_PDKeyAreaRAPSSta_enum]
  [task_time_s] -> WasherWiper/1(task_time_s)
  VINP_SenstivityPosition_enum/1 -> CSW/19(VINP_SenstivityPosition_enum)
  CSW/8(VBCM_SenstivityPosnCmd_enum) -> VBCM_SenstivityPosnCmd_enum/1
  VINP_FlashAutoUnlock_enum/1 -> Personal_Setting/70(VINP_FlashAutoUnlock_enum)
  VINP_ADASACCSta_enum/1 -> Personal_Setting/66(VINP_ADASACCSta_enum)
  VINP_IVIDrivingLockSWSta_flg/1 -> Personal_Setting/69(VINP_IVIDrivingLockSWSta_flg)
  VINP_IVIStoppingUnlockSWSta_flg/1 -> Personal_Setting/67(VINP_IVIStoppingUnlockSWSta_flg)
  VINP_SWC2LRightSta_flg/1 -> Personal_Setting/63(VINP_SWC2LRightSta_flg)
  VINP_FlashAutoLock_enum/1 -> Personal_Setting/68(VINP_FlashAutoLock_enum)
  VINP_FDCVMCSpdCtrlModeSta_enum/1 -> Personal_Setting/65(VINP_FDCVMCSpdCtrlModeSta_enum)
  VINP_SWC2LLeftSta_flg/1 -> Personal_Setting/64(VINP_SWC2LLeftSta_flg)
  VINP_FlashACCLevelSta57_enum/1 -> Personal_Setting/62(VINP_FlashACCLevelSta57_enum)
  VINP_FlashACCLevelSta34_enum/1 -> Personal_Setting/61(VINP_FlashACCLevelSta34_enum)
  VINP_TimeGapLevel_enum/1 -> Personal_Setting/59(VINP_TimeGapLevel_enum)
  VINP_FlashACCLevelSta12_enum/1 -> Personal_Setting/60(VINP_FlashACCLevelSta12_enum)
  VINP_PTGIsSetHeight_flg/1 -> Personal_Setting/50(VINP_PTGIsSetHeight_flg)
  Personal_Setting/63(VBCM_AutoUnlockSta_flg) -> [VBCM_AutoUnlockSta_flg]  "VBCM_AutoUnlockSta_flg"
  Personal_Setting/61(VBCM_AutoLockSta_flg) -> [VBCM_AutoLockSta_flg]  "VBCM_AutoLockSta_flg"
  Personal_Setting/55(VBCM_TimeGapLevelSta_enum) -> VBCM_TimeGapLevelSta_enum/1  "VBCM_TimeGapLevelSta_enum"
  Personal_Setting/56(VBCM_ACCLevelMem12_enum) -> VBCM_ACCLevelMem12_enum/1  "VBCM_ACCLevelMem12_enum"
  Personal_Setting/57(VBCM_ACCLevelMem34_enum) -> VBCM_ACCLevelMem34_enum/1  "VBCM_ACCLevelMem34_enum"
  Personal_Setting/58(VBCM_ACCLevelMem57_enum) -> VBCM_ACCLevelMem57_enum/1  "VBCM_ACCLevelMem57_enum"
  Personal_Setting/59(VBCM_LRightStaCmd_flg) -> VBCM_LRightStaCmd_flg/1  "VBCM_LRightStaCmd_flg"
  Personal_Setting/60(VBCM_LLeftStaCmd_flg) -> VBCM_LLeftStaCmd_flg/1  "VBCM_LLeftStaCmd_flg"
  Personal_Setting/62(VBCM_AutoLockMem_enum) -> VBCM_AutoLockMem_enum/1  "VBCM_AutoLockMem_enum"
  Personal_Setting/64(VBCM_AutoUnlockMem_enum) -> VBCM_AutoUnlockMem_enum/1  "VBCM_AutoUnlockMem_enum"
  VINP_CANMsgValidBodyZonePS1_flg/1 -> Personal_Setting/71(VINP_CANMsgValidBodyZonePS1_flg)
  [VINP_DiagFMHT_s] -> DID Judgement/1(VINP_DiagFMHT_s)
  DID Judgement/2(VBCM_DiagFLTC_mA) -> [VBCM_DiagFLTC_mA]
  DID Judgement/6(VBCM_DiagDRLOFF_flg) -> [VBCM_DiagDRLOFF_flg]
  DID Judgement/1(VBCM_DiagFMHT_s) -> [VBCM_DiagFMHT_s]
  DID Judgement/5(VBCM_DiagRRTC_mA) -> [VBCM_DiagRRTC_mA]
  DID Judgement/4(VBCM_DiagRLTC_mA) -> [VBCM_DiagRLTC_mA]
  DID Judgement/3(VBCM_DiagFRTC_mA) -> [VBCM_DiagFRTC_mA]
  [VBCM_DiagFLTC_mA] -> FlasherSignal/16(VBCM_DiagFLTC_mA)
  [VBCM_DiagFRTC_mA] -> FlasherSignal/17(VBCM_DiagFRTC_mA)
  [VBCM_DiagRRTC_mA] -> FlasherSignal/19(VBCM_DiagRRTC_mA)
  [VBCM_DiagRLTC_mA] -> FlasherSignal/18(VBCM_DiagRLTC_mA)
  VINP_funAuto_flg/1 -> Terminator/1
  Ground/1 -> CenterDoorLock/12(VINP_funAuto_flg)
  [VBCM_TurnLPErrEN_flg] -> FlasherSignal/38(VBCM_TurnLPErrEN_flg)
  DID Judgement/7(VBCM_TurnLPErrEN_flg) -> [VBCM_TurnLPErrEN_flg]
  [VBCM_DiagDRLOFF_flg] -> ExteriorLight/21(VINP_DiagDRLOFF_flg)
  [VBCM_DiagFMHT_s] -> ExteriorLight/22(VINP_DiagFMHT_s)
  VINP_DiagWipRLSCmdCutEN_flg/1 -> WasherWiper/16(VINP_DiagWipRLSCmdCutEN_flg)
  VINP_DiagRLSCmdCutTime_s/1 -> WasherWiper/17(VINP_DiagRLSCmdCutTime_s)
  VINP_DiagWipRLSCmdHoldEN_flg/1 -> WasherWiper/18(VINP_DiagWipRLSCmdHoldEN_flg)
  VINP_DiagRLSCmdHoldTime_s/1 -> WasherWiper/19(VINP_DiagRLSCmdHoldTime_s)
  VINP_LeftHallPos_cnt/1 -> Personal_Setting/72(VINP_LeftHallPos_cnt)
  VINP_VehicleType_enum/1 -> [VINP_VehicleType_enum]
  [VINP_VehicleType_enum] -> Amb/27(VINP_VehicleType_enum)
  [VINP_VehicleType_enum] -> FlasherSignal/39(VINP_VehicleType_enum)
  [VINP_VehicleType_enum] -> PTG/17(VINP_VehicleType_enum)
  [VINP_VehicleType_enum] -> Personal_Setting/73(VINP_VehicleType_enum)
  HMI_Custom_Button/1(VBCM_HMIKey1FuncSta_enum) -> VBCM_HMIKey1FuncSta_enum/1  "VBCM_HMIKey1FuncSta_enum"
  HMI_Custom_Button/2(VBCM_HMIKey2FuncSta_enum) -> VBCM_HMIKey2FuncSta_enum/1  "VBCM_HMIKey2FuncSta_enum"
  HMI_Custom_Button/3(VBCM_HMIKey3FuncSta_enum) -> VBCM_HMIKey3FuncSta_enum/1  "VBCM_HMIKey3FuncSta_enum"
  HMI_Custom_Button/4(VBCM_HMIKey4FuncSta_enum) -> VBCM_HMIKey4FuncSta_enum/1  "VBCM_HMIKey4FuncSta_enum"
  HMI_Custom_Button/5(VBCM_HMIKey5FuncSta_enum) -> VBCM_HMIKey5FuncSta_enum/1  "VBCM_HMIKey5FuncSta_enum"
  HMI_Custom_Button/6(VBCM_HMIKey6FuncSta_enum) -> VBCM_HMIKey6FuncSta_enum/1  "VBCM_HMIKey6FuncSta_enum"
  HMI_Custom_Button/7(VBCM_HMIKey7FuncSta_enum) -> VBCM_HMIKey7FuncSta_enum/1  "VBCM_HMIKey7FuncSta_enum"
  HMI_Custom_Button/8(VBCM_HMIKey8FuncSta_enum) -> VBCM_HMIKey8FuncSta_enum/1  "VBCM_HMIKey8FuncSta_enum"
  VINP_IVIHMICustmiKEYSta_enum/1 -> HMI_Custom_Button/1(VINP_IVIHMICustmiKEYSta_enum)
  VINP_IVIHMICustmiFunSta_enum/1 -> HMI_Custom_Button/2(VINP_IVIHMICustmiFunSta_enum)
  VINP_FlashHMIKey1Func_enum/1 -> HMI_Custom_Button/3(VINP_FlashHMIKey1Func_enum)
  VINP_FlashHMIKey2Func_enum/1 -> HMI_Custom_Button/4(VINP_FlashHMIKey2Func_enum)
  VINP_FlashHMIKey3Func_enum/1 -> HMI_Custom_Button/5(VINP_FlashHMIKey3Func_enum)
  VINP_FlashHMIKey4Func_enum/1 -> HMI_Custom_Button/6(VINP_FlashHMIKey4Func_enum)
  VINP_FlashHMIKey5Func_enum/1 -> HMI_Custom_Button/7(VINP_FlashHMIKey5Func_enum)
  VINP_FlashHMIKey6Func_enum/1 -> HMI_Custom_Button/8(VINP_FlashHMIKey6Func_enum)
  VINP_FlashHMIKey7Func_enum/1 -> HMI_Custom_Button/9(VINP_FlashHMIKey7Func_enum)
  VINP_FlashHMIKey8Func_enum/1 -> HMI_Custom_Button/10(VINP_FlashHMIKey8Func_enum)
  WasherWiper/6(VBCM_AutoWipHSpdENSta_flg) -> VBCM_AutoWipHSpdENSta_flg/1  "VBCM_AutoWipHSpdENSta_flg"
  VINP_FlashAutoWipHSpdEN_flg/1 -> WasherWiper/20(VINP_FlashAutoWipHSpdEN_flg)
  VINP_IVIAutoWipHSpdSWCmd_flg/1 -> WasherWiper/21(VINP_IVIAutoWipHSpdSWCmd_flg)
  VINP_SWC2RCustomizeSta_flg/1 -> Personal_Setting/74(VINP_SWC2RCustomizeSta_flg)
  VINP_IVISWCRUndefinedSta_enum/1 -> Personal_Setting/75(VINP_IVISWCRUndefinedSta_enum)
  VINP_HMIAutoInterLightCmd_flg/1 -> Personal_Setting/76(VINP_HMIAutoInterLightCmd_flg)
  [task_time_s] -> PTG/1(task_time_s)
  VINP_IVISnowModeCmd_flg/1 -> Amb/28(VINP_IVISnowModeCmd_flg)
  [VINP_DrDoorSW_flg] -> Amb/29(VINP_DrDoorSW_flg)
  [VINP_PsDoorSW_flg] -> Amb/30(VINP_PsDoorSW_flg)
  [VINP_RLDoorSW_flg] -> Amb/31(VINP_RLDoorSW_flg)
  [VINP_RRDoorSW_flg] -> Amb/32(VINP_RRDoorSW_flg)
  [VBCM_HornCtrl_flg] -> VBCM_HornCtrl_flg/1
  [VBCM_AllDoorSW_flg] -> VBCM_AllDoorSW_flg/1
  [VBCM_BCMDoorLockSta_flg] -> VBCM_BCMDoorLockSta_flg/1
  [VBCM_HoodSW_flg] -> VBCM_HoodSW_flg/1
  [VBCM_TailgateSW_flg] -> VBCM_TailgateSW_flg/1
  [VBCM_PosLamp_flg] -> VBCM_PosLamp_flg/1
  [VBCM_LBSD_flg] -> VBCM_LBSD_flg/1
  [VBCM_RBSD_flg] -> VBCM_RBSD_flg/1
  [VBCM_LTurnLP_flg] -> VBCM_LTurnLP_flg/1
  [VBCM_RTurnLP_flg] -> VBCM_RTurnLP_flg/1
  [VBCM_SPTGDet_flg] -> VBCM_SPTGDet_flg/1
  [VBCM_APSOpenPTG_flg] -> VBCM_APSOpenPTG_flg/1
  [VBCM_ATCtrl_enum] -> VBCM_ATCtrl_enum/1
  [FDC_BCM_AmbFunEN_Sta] -> VBCM_AmbFunEN_flg/1
  [FDC_BCM_AmbWelEN_Sta] -> VBCM_AmbWelEN_flg/1
  [FDC_BCM_AmbDimEN_Sta] -> VBCM_AmbDimEN_flg/1
  [FDC_BCM_AmbLinkDriSta_Sta] -> VBCM_AmbLinkDriSta_flg/1
  [FDC_BCM_AmbPwrWarnEN_Sta] -> VBCM_AmbPwrWarnEN_flg/1
  [FDC_BCM_AmbODAEN_Sta] -> VBCM_AmbODAEN_flg/1
  [FDC_BCM_AmbColorSta_Sta] -> VBCM_AmbColorSta_enum/1
  [FDC_BCM_AmbBrightSta_Sta] -> VBCM_AmbBrightSta_enum/1
  [VBCM_LBeam_flg] -> VBCM_LBeam_flg/1
  [VBCM_DimSwSta_flg] -> VBCM_DimSwSta_flg/1  "VBCM_DimSwSta_flg"
  [VBCM_PassSWSta_flg] -> VBCM_PassSWSta_flg/1  "VBCM_PassSWSta_flg"
  [VBCM_FWipSwSta_enum] -> VBCM_FWipSwSta_enum/1  "VBCM_FWipSwSta_enum"
  [VBCM_FWasSwSta_enum] -> VBCM_FWasSwSta_enum/1  "VBCM_FWasSwSta_enum"
  [VBCM_TurnSwSta_enum] -> VBCM_TurnSwSta_enum/1  "VBCM_TurnSwSta_enum"
  [VBCM_SPTGENFun_flg] -> VBCM_SPTGENFun_flg/1  "VBCM_SPTGENFun_flg"
  [VBCM_OutMode_enum] -> VBCM_OutMode_enum/1
  [VBCM_TurnSwTSetSta_enum] -> VBCM_TurnSwTSetSta_enum/1
  [VBCM_DoorLockIND_flg] -> VBCM_DoorLockIND_flg/1
  [VBCM_CTDLockSW_flg] -> VBCM_CTDLockSW_flg/1
  [VBCM_MirrorCtrl_enum] -> VBCM_MirrorCtrl_enum/1
  [VBCM_RoomLampH_flg] -> VBCM_RoomLampH_flg/1
  [VBCM_TailgateHDSW_flg] -> VBCM_TailgateHDSW_flg/1
  [VBCM_LockSetting_flg] -> VBCM_LockSetting_flg/1
  [FDC_BCM_WalkInUnLkEnFun_Sta] -> VBCM_WalkInUnLkEnFunSta_flg/1
  [FDC_BCM_WalkOutLkEnFun_Sta] -> VBCM_WalkOutLkEnFunSta_flg/1
  [FDC_BCM_RmLpModeENFun_Sta] -> VBCM_RmLpModeENFunSta_flg/1
  [FDC_BCM_FollowMeENFun_Sta] -> VBCM_FollowMeENFunSta_flg/1
  [VBCM_AutoLockSta_flg] -> VBCM_AutoLockSta_flg/1
  [VBCM_AutoUnlockSta_flg] -> VBCM_AutoUnlockSta_flg/1
  Unit Delay1/1 -> [BCMInitial]
  [VINP_DiagFLTC_mA] -> DID Judgement/2(VINP_DiagFLTC_mA)
  [VINP_DiagFRTC_mA] -> DID Judgement/3(VINP_DiagFRTC_mA)
  [VINP_DiagRLTC_mA] -> DID Judgement/4(VINP_DiagRLTC_mA)
  [VINP_DiagRRTC_mA] -> DID Judgement/5(VINP_DiagRRTC_mA)
  [VINP_DiagDRLOFF_flg] -> DID Judgement/6(VINP_DiagDRLOFF_flg)
  [VINP_VehicleType_enum] -> DID Judgement/7(VINP_VehicleType_enum)
  VINP_LDrvControlCommand_pct/1 -> [VINP_LDrvControlCommand_pct]
  VINP_LPasControlCommand_pct/1 -> [VINP_LPasControlCommand_pct]
  VINP_LRLDControlCommand_pct/1 -> [VINP_LRLDControlCommand_pct]
  VINP_LRRDControlCommand_pct/1 -> [VINP_LRRDControlCommand_pct]
  [VINP_VehicleType_enum] -> Vehicle Type Diff Fun/1(VINP_VehicleType_enum)
  Vehicle Type Diff Fun/1(VBCM_APMDoorCtrlEN_flg) -> [VBCM_APMDoorCtrlEN_flg]
  [VBCM_APMDoorCtrlEN_flg] -> Window_Control_Sig_Combine/1(VBCM_APMDoorCtrlEN_flg)
  Vehicle Type Diff Fun/2(VBCM_RightHandDriveEN_flg) -> [VBCM_RightHandDriveEN_flg]
  [VBCM_RightHandDriveEN_flg] -> Window_Control_Sig_Combine/2(VBCM_RightHandDriveEN_flg)
  [VINP_LDrvControlCommand_pct] -> Window_Control_Sig_Combine/6(VINP_LDrvControlCommand_pct)
  [VINP_LPasControlCommand_pct] -> Window_Control_Sig_Combine/10(VINP_LPasControlCommand_pct)
  [VINP_LRLDControlCommand_pct] -> Window_Control_Sig_Combine/14(VINP_LRLDControlCommand_pct)
  [VINP_LRRDControlCommand_pct] -> Window_Control_Sig_Combine/18(VINP_LRRDControlCommand_pct)
  VINP_DKCDrvWdwCtrlCmd_pct/1 -> Window_Control_Sig_Combine/3(VINP_DKCDrvWdwCtrlCmd_pct)
  VINP_ConnDrvWdwCtrlCmd_pct/1 -> Window_Control_Sig_Combine/4(VINP_ConnDrvWdwCtrlCmd_pct)
  VINP_DKCPasWdwCtrlCmd_pct/1 -> Window_Control_Sig_Combine/7(VINP_DKCPasWdwCtrlCmd_pct)
  VINP_ConnPasWdwCtrlCmd_pct/1 -> Window_Control_Sig_Combine/8(VINP_ConnPasWdwCtrlCmd_pct)
  VINP_DKCRLDWdwCtrlCmd_pct/1 -> Window_Control_Sig_Combine/11(VINP_DKCRLDWdwCtrlCmd_pct)
  VINP_ConnRLDWdwCtrlCmd_pct/1 -> Window_Control_Sig_Combine/12(VINP_ConnRLDWdwCtrlCmd_pct)
  VINP_DKCRRDWdwCtrlCmd_pct/1 -> Window_Control_Sig_Combine/15(VINP_DKCRRDWdwCtrlCmd_pct)
  VINP_ConnRRDWdwCtrlCmd_pct/1 -> Window_Control_Sig_Combine/16(VINP_ConnRRDWdwCtrlCmd_pct)
  Window_Control_Sig_Combine/1(VBCM_DrvWdwCtrlCmd_pct) -> VBCM_DrvWdwCtrlCmd_pct/1  "VBCM_DrvWdwCtrlCmd_pct"
  Window_Control_Sig_Combine/2(VBCM_DrvWdwReqAP_enum) -> VBCM_DrvWdwReqAP_enum/1  "VBCM_DrvWdwReqAP_enum"
  Window_Control_Sig_Combine/3(VBCM_PasWdwCtrlCmd_pct) -> VBCM_PasWdwCtrlCmd_pct/1  "VBCM_PasWdwCtrlCmd_pct"
  Window_Control_Sig_Combine/4(VBCM_PasWdwReqAP_enum) -> VBCM_PasWdwReqAP_enum/1  "VBCM_PasWdwReqAP_enum"
  Window_Control_Sig_Combine/5(VBCM_DrRWdwCtrlCmd_pct) -> VBCM_DrRWdwCtrlCmd_pct/1  "VBCM_DrRWdwCtrlCmd_pct"
  Window_Control_Sig_Combine/6(VBCM_DrRWdwReqAP_enum) -> VBCM_DrRWdwReqAP_enum/1  "VBCM_DrRWdwReqAP_enum"
  Window_Control_Sig_Combine/7(VBCM_PsRWdwCtrlCmd_pct) -> VBCM_PsRWdwCtrlCmd_pct/1  "VBCM_PsRWdwCtrlCmd_pct"
  Window_Control_Sig_Combine/8(VBCM_PsRWdwReqAP_enum) -> VBCM_PsRWdwReqAP_enum/1  "VBCM_PsRWdwReqAP_enum"
  [task_time_s] -> APM_Door/1(task_time_s)
  [VINP_LDrvControlCommand_pct] -> APM_Door/3(VINP_LDrvControlCommand_pct)
  [VINP_DrDoorSW_flg] -> APM_Door/5(VINP_DrDoorSW_flg)
  [VINP_LPasControlCommand_pct] -> APM_Door/6(VINP_LPasControlCommand_pct)
  [VINP_PsDoorSW_flg] -> APM_Door/8(VINP_PsDoorSW_flg)
  [VINP_LRLDControlCommand_pct] -> APM_Door/9(VINP_LRLDControlCommand_pct)
  [VINP_RLDoorSW_flg] -> APM_Door/11(VINP_RLDoorSW_flg)
  [VINP_LRRDControlCommand_pct] -> APM_Door/12(VINP_LRRDControlCommand_pct)
  [VINP_RRDoorSW_flg] -> APM_Door/14(VINP_RRDoorSW_flg)
  [BCMInitial] -> APM_Door/16(BCMInitial)
  [VINP_CANMsgValidIVI2_flg] -> APM_Door/17(VINP_CANMsgValidIVI2_flg)
  [VINP_CANMsgValidGWZoneDR1_flg] -> APM_Door/18(VINP_CANMsgValidGWZoneDR1_flg)
  [VINP_CANMsgValidGWZoneFR1_flg] -> APM_Door/19(VINP_CANMsgValidGWZoneFR1_flg)
  VINP_OpenDrOpenWdoSW_flg/1 -> APM_Door/2(VINP_OpenDrOpenWdoSW_flg)
  VINP_LDrvValWdwOpened_pct/1 -> APM_Door/4(VINP_LDrvValWdwOpened_pct)
  VINP_LPasValWdwOpened_pct/1 -> APM_Door/7(VINP_LPasValWdwOpened_pct)
  VINP_LRLDValWdwOpened_pct/1 -> APM_Door/10(VINP_LRLDValWdwOpened_pct)
  VINP_LRRDValWdwOpened_pct/1 -> APM_Door/13(VINP_LRRDValWdwOpened_pct)
  VINP_FlashAPMDoorControlSta_flg/1 -> APM_Door/15(VINP_FlashAPMDoorControlSta_flg)
  VINP_CANMsgValidzGWLINDr1_flg/1 -> APM_Door/20(VINP_CANMsgValidzGWLINDr1_flg)
  APM_Door/2(VBCM_LDrvCtrlCmd_pct) -> [VBCM_LDrvCtrlCmd_pct]
  APM_Door/3(VBCM_LPasCtrlCmd_pct) -> [VBCM_LPasCtrlCmd_pct]
  APM_Door/4(VBCM_LRLDCtrlCmd_pct) -> [VBCM_LRLDCtrlCmd_pct]
  APM_Door/5(VBCM_LRRDCtrlCmd_pct) -> [VBCM_LRRDCtrlCmd_pct]
  [VBCM_BCMPasWdwCtrlCmd_pct] -> Window_Control_Sig_Combine/9(VBCM_BCMPasWdwCtrlCmd_pct)
  [VBCM_BCMRLDWdwCtrlCmd_pct] -> Window_Control_Sig_Combine/13(VBCM_BCMRLDWdwCtrlCmd_pct)
  [VBCM_BCMRRDWdwCtrlCmd_pct] -> Window_Control_Sig_Combine/17(VBCM_BCMRRDWdwCtrlCmd_pct)
  [VBCM_BCMDrvWdwCtrlCmd_pct] -> Window_Control_Sig_Combine/5(VBCM_BCMDrvWdwCtrlCmd_pct)
  BCM_Window_Control/1(VBCM_BCMDrvWdwCtrlCmd_pct) -> [VBCM_BCMDrvWdwCtrlCmd_pct]
  BCM_Window_Control/2(VBCM_BCMPasWdwCtrlCmd_pct) -> [VBCM_BCMPasWdwCtrlCmd_pct]
  BCM_Window_Control/3(VBCM_BCMRLDWdwCtrlCmd_pct) -> [VBCM_BCMRLDWdwCtrlCmd_pct]
  BCM_Window_Control/4(VBCM_BCMRRDWdwCtrlCmd_pct) -> [VBCM_BCMRRDWdwCtrlCmd_pct]
  [VBCM_APMDoorCtrlEN_flg] -> BCM_Window_Control/1(VBCM_APMDoorCtrlEN_flg)
  [VBCM_AntitheftSta_enum] -> BCM_Window_Control/2(VBCM_AntitheftSta_enum)
  VINP_OFFACMode_enum/1 -> BCM_Window_Control/3(VINP_OFFACMode_enum)
  [VBCM_CLWinLockDrSta_flg] -> BCM_Window_Control/4(VBCM_CLWinLockDrSta_flg)
  [VBCM_LPasCtrlCmd_pct] -> BCM_Window_Control/6(VBCM_LPasCtrlCmd_pct)
  [VBCM_LRLDCtrlCmd_pct] -> BCM_Window_Control/7(VBCM_LRLDCtrlCmd_pct)
  [VBCM_LRRDCtrlCmd_pct] -> BCM_Window_Control/8(VBCM_LRRDCtrlCmd_pct)
  [VBCM_LDrvCtrlCmd_pct] -> BCM_Window_Control/5(VBCM_LDrvCtrlCmd_pct)
  Personal_Setting/65(VBCM_CLWinLockDrSta_flg) -> [VBCM_CLWinLockDrSta_flg]
  VINP_IVICLWinLockDrSW_flg/1 -> Personal_Setting/77(VINP_IVICLWinLockDrSW_flg)
  VINP_FlashCLWinLockDrSta_enum/1 -> Personal_Setting/78(VINP_FlashCLWinLockDrSta_enum)
  Personal_Setting/66(VBCM_CLWinLockDrStaMem_enum) -> VBCM_CLWinLockDrStaMem_enum/1
  [VINP_IVICarWashModeCmd_flg] -> PowerMirror/9(VINP_IVICarWashModeCmd_flg)
  VINP_IVIMirrorFoldedSWSta_flg/1 -> [VINP_IVIMirrorFoldedSWSta_flg]
  [VINP_IVIMirrorFoldedSWSta_flg] -> PowerMirror/10(VINP_IVIMirrorFoldedSWSta_flg)
  [VINP_IVICarWashModeCmd_flg] -> WasherWiper/22(VINP_IVICarWashModeCmd_flg)
  [VINP_IVICarWashModeCmd_flg] -> Personal_Setting/79(VINP_IVICarWashModeCmd_flg)
  [VINP_IVICarWashModeCmd_flg] -> BCM_Window_Control/9(VINP_IVICarWashModeCmd_flg)
  Vehicle Type Diff Fun/3(VBCM_HLBeamENPwrSta_enum) -> [VBCM_HLBeamENPwrSta_enum]
  Vehicle Type Diff Fun/4(VBCM_showupEN_flg) -> [VBCM_showupEN_flg]
  [VBCM_HLBeamENPwrSta_enum] -> ExteriorLight/24(VBCM_HLBeamENPwrSta_enum)
  [VBCM_showupEN_flg] -> ExteriorLight/25(VBCM_showupEN_flg)
  [VBCM_CLWinLockDrSta_flg] -> VBCM_CLWinLockDrSta_flg/1
  VINP_WlcmLightMode_enum/1 -> Vehicle Type Diff Fun/2(VINP_WlcmLightMode_enum)
  [VPMM_PwrSta_enum] -> Vehicle Type Diff Fun/3(VPMM_PwrSta_enum)
  Vehicle Type Diff Fun/5(VBCM_UnlockWelcomeEN_flg) -> [VBCM_UnlockWelcomeEN_flg]
  [VBCM_UnlockWelcomeEN_flg] -> FlasherSignal/40(VBCM_UnlockWelcomeEN_flg)
  ExteriorLight/12(VBCM_showup_flg) -> Terminator1/1
  VINP_PDKeyWelcome_enum/1 -> Terminator2/1
  Window_Control_Sig_Combine/9(VBCM_WinLFOpenedSta_pct) -> VBCM_WinLFOpenedSta_pct/1  "VBCM_WinLFOpenedSta_pct"
  Window_Control_Sig_Combine/10(VBCM_WinRFOpenedSta_pct) -> VBCM_WinRFOpenedSta_pct/1  "VBCM_WinRFOpenedSta_pct"
  Window_Control_Sig_Combine/11(VBCM_WinLROpenedSta_pct) -> VBCM_WinLROpenedSta_pct/1  "VBCM_WinLROpenedSta_pct"
  Window_Control_Sig_Combine/12(VBCM_WinRROpenedSta_pct) -> VBCM_WinRROpenedSta_pct/1  "VBCM_WinRROpenedSta_pct"
  VINP_BDAPMWinFOpenedSta_pct/1 -> Window_Control_Sig_Combine/19(VINP_BDWinFOpenedSta_pct)
  VINP_BDAPMWinROpenedSta_pct/1 -> Window_Control_Sig_Combine/20(VINP_BDWinROpenedSta_pct)
  VINP_BPAPMWinFOpenedSta_pct/1 -> Window_Control_Sig_Combine/21(VINP_BPWinFOpenedSta_pct)
  VINP_BPAPMWinROpenedSta_pct/1 -> Window_Control_Sig_Combine/22(VINP_BPWinROpenedSta_pct)
  VINP_SRRODAWarnL_enum/1 -> [VINP_SRRODAWarnL_enum]
  VINP_SRRODAWarnR_enum/1 -> [VINP_SRRODAWarnR_enum]
  [VINP_CANMsgValidIVI2_flg] -> Switch/2
  VINP_IVICarWashModeCmd_flg/1 -> Switch/1
  Unit Delay3/1 -> Data Type Conversion2/1
  VTQD_CrashDetd_flg/1 -> [VTQD_CrashDetd_flg]
  [VTQD_CrashDetd_flg] -> CenterDoorLock/15(VTQD_CrashDetd_flg)
  [VTQD_CrashDetd_flg] -> FoxtronPiOutput/1(VTQD_CrashDetd_flg)
  [VINP_DrLockSta_flg] -> FoxtronPiOutput/2(VINP_DrLockSta_flg)
  [VINP_DrLockSta_flg] -> AntiTheft/9(VINP_DrLockSta_flg)
  VINP_DrLockSta_flg/1 -> [VINP_DrLockSta_flg]
  [VBCM_AllDoorSW_flg] -> FoxtronPiOutput/3(VBCM_AllDoorSW_flg)
  AntiTheft/12(VBCM_DrDoorSW_flg) -> [VBCM_DrDoorSW_flg]
  AntiTheft/15(VBCM_RRDoorSW_flg) -> [VBCM_RRDoorSW_flg]
  AntiTheft/14(VBCM_RLDoorSW_flg) -> [VBCM_RLDoorSW_flg]
  AntiTheft/13(VBCM_PsDoorSW_flg) -> [VBCM_PsDoorSW_flg]
  [VBCM_DrDoorSW_flg] -> VBCM_DrDoorSW_flg/1
  [VBCM_PsDoorSW_flg] -> VBCM_PsDoorSW_flg/1
  [VBCM_RLDoorSW_flg] -> VBCM_RLDoorSW_flg/1
  [VBCM_RRDoorSW_flg] -> VBCM_RRDoorSW_flg/1
  [VINP_DrDoorSW_flg] -> FoxtronPiOutput/4(VINP_DrDoorSW_flg)
  [VINP_PsDoorSW_flg] -> FoxtronPiOutput/5(VINP_PsDoorSW_flg)
  [VINP_RLDoorSW_flg] -> FoxtronPiOutput/6(VINP_RLDoorSW_flg)
  [VINP_RRDoorSW_flg] -> FoxtronPiOutput/7(VINP_RRDoorSW_flg)
  [VINP_TailgateSW_flg] -> FoxtronPiOutput/8(VINP_TailgateSW_flg)
  [VINP_HoodSW_flg] -> AntiTheft/3(VINP_HoodSW_flg)
  VINP_HoodSW_flg/1 -> [VINP_HoodSW_flg]
  [VINP_HoodSW_flg] -> FoxtronPiOutput/9(VINP_HoodSW_flg)
  [VBCM_TurnSwSta_enum] -> FoxtronPiOutput/10(VBCM_TurnSwSta_enum)
  [VBCM_DimSwSta_flg] -> FoxtronPiOutput/11(VBCM_DimSwSta_flg)
  [VBCM_PassSWSta_flg] -> FoxtronPiOutput/12(VBCM_PassSWSta_flg)
  [VBCM_PosLamp_flg] -> FoxtronPiOutput/13(VBCM_PosLamp_flg)
  [VBCM_LBeam_flg] -> FoxtronPiOutput/14(VBCM_LBeam_flg)
  [VBCM_HBeam_flg] -> VBCM_HBeam_flg/1
  [VBCM_RrFogLamp_flg] -> VBCM_RrFogLamp_flg/1
  [VBCM_BrakeLamp_flg] -> VBCM_BrakeLamp_flg/1
  [VBCM_ReverseLamp_flg] -> VBCM_ReverseLamp_flg/1
  [VBCM_LDRL_flg] -> VBCM_LDRL_flg/1
  [VBCM_RDRL_flg] -> VBCM_RDRL_flg/1
  [VBCM_HBeam_flg] -> FoxtronPiOutput/15(VBCM_HBeam_flg)
  [VBCM_RDRL_flg] -> FoxtronPiOutput/16(VBCM_RDRL_flg)
  [VBCM_LDRL_flg] -> FoxtronPiOutput/17(VBCM_LDRL_flg)
  [VBCM_LTurnLP_flg] -> FoxtronPiOutput/18(VBCM_LTurnLP_flg)
  [VBCM_RTurnLP_flg] -> FoxtronPiOutput/19(VBCM_RTurnLP_flg)
  [VBCM_BrakeLamp_flg] -> FoxtronPiOutput/20(VBCM_BrakeLamp_flg)
  [VBCM_ReverseLamp_flg] -> FoxtronPiOutput/21(VBCM_ReverseLamp_flg)
  [VBCM_RrFogLamp_flg] -> FoxtronPiOutput/22(VBCM_RrFogLamp_flg)
  Switch1/1 -> [VBCM_PosLamp_flg]  "VBCM_PosLamp_flg"
  Switch2/1 -> [VBCM_LBeam_flg]  "VBCM_LBeam_flg"
  VINP_FoxPiPosLampCtrlEN_flg/1 -> Switch1/2
  VINP_FoxPiPosLampCtrl_flg/1 -> Switch1/1
  ExteriorLight/1(VBCM_PosLamp_flg) -> Switch1/3
  ExteriorLight/2(VBCM_LBeam_flg) -> Switch2/3
  VBCM_FoxPiLBeamCtrl_flg/1 -> Switch2/1
  VBCM_FoxPiLBeamCtrlEN_flg/1 -> Switch2/2
  ExteriorLight/3(VBCM_HBeam_flg) -> Switch3/3
  Switch3/1 -> [VBCM_HBeam_flg]  "VBCM_HBeam_flg"
  VBCM_FoxPiHBeamCtrl_flg/1 -> Switch3/1
  VBCM_FoxPiHBeamCtrlEN_flg/1 -> Switch3/2
  ExteriorLight/8(VBCM_RDRL_flg) -> Switch4/3
  Switch4/1 -> [VBCM_RDRL_flg]  "VBCM_RDRL_flg"
  VBCM_FoxPiRDRLCtrl_flg/1 -> Switch4/1
  VBCM_FoxPiRDRLCtrlEN_flg/1 -> Switch4/2
  Switch5/1 -> [VBCM_LDRL_flg]  "VBCM_LDRL_flg"
  ExteriorLight/7(VBCM_LDRL_flg) -> Switch5/3
  VBCM_FoxPiLDRLCtrl_flg/1 -> Switch5/1
  VBCM_FoxPiLDRLCtrlEN_flg/1 -> Switch5/2
  VBCM_FoxPiLTurnLPCtrl_flg/1 -> Switch6/1
  VBCM_FoxPiLTurnLPCtrlEN_flg/1 -> Switch6/2
  Switch6/1 -> [VBCM_LTurnLP_flg]  "VBCM_LTurnLP_flg"
  FlasherSignal/2(VBCM_LTurnLP_flg) -> Switch6/3
  FlasherSignal/3(VBCM_RTurnLP_flg) -> Switch7/3
  Switch7/1 -> [VBCM_RTurnLP_flg]  "VBCM_RTurnLP_flg"
  VBCM_FoxPiRTurnLPCtrl_flg/1 -> Switch7/1
  VBCM_FoxPiRTurnLPCtrlEN_flg/1 -> Switch7/2
  ExteriorLight/6(VBCM_ReverseLamp_flg) -> Switch8/3
  Switch8/1 -> [VBCM_ReverseLamp_flg]  "VBCM_ReverseLamp_flg"
  ExteriorLight/4(VBCM_RrFogLamp_flg) -> Switch9/3
  Switch9/1 -> [VBCM_RrFogLamp_flg]  "VBCM_RrFogLamp_flg"
  ExteriorLight/5(VBCM_BrakeLamp_flg) -> Switch10/3
  Switch10/1 -> [VBCM_BrakeLamp_flg]  "VBCM_BrakeLamp_flg"
  VBCM_FoxPiBkLampCtrl_flg/1 -> Switch10/1
  VBCM_FoxPiBkLampCtrlEN_flg/1 -> Switch10/2
  VBCM_FoxPiRevCtrl_flg/1 -> Switch8/1
  VBCM_FoxPiRevCtrlEN_flg/1 -> Switch8/2
  VBCM_FoxPiRrFogLpCtrl_flg/1 -> Switch9/1
  VBCM_FoxPiRrFogLpCtrlEN_flg/1 -> Switch9/2
  VINP_FoxPiAmbColorCtrl_enum/1 -> Amb/37(VINP_FoxPiAmbColorCtrl_enum)
  VINP_FoxPiAmbCtrlEN_flg/1 -> Amb/33(VINP_FoxPiAmbCtrlEN_flg)
  VINP_FoxPiAmbBreathCtrl_enum/1 -> Amb/34(VINP_FoxPiAmbBreathCtrl_enum)
  VINP_FoxPiAmbAreaCtrl_enum/1 -> Amb/35(VINP_FoxPiAmbAreaCtrl_enum)
  VINP_FoxPiAmbBrightCtrl_enum/1 -> Amb/36(VINP_FoxPiAmbBrightCtrl_enum)
  FoxtronPiOutput/1(VBCM_FoxPiSwitchSta_enum) -> VBCM_FoxPiSwitchSta_enum/1  "VBCM_FoxPiSwitchSta_enum"
  FoxtronPiOutput/2(VBCM_FoxPiLampSta_enum) -> VBCM_FoxPiLampSta_enum/1  "VBCM_FoxPiLampSta_enum"
  Data Type Conversion1/1 -> Unit Delay3/1, [VINP_IVICarWashModeCmd_flg]
  Switch/1 -> Data Type Conversion1/1
  Data Type Conversion2/1 -> Switch/3
